simulink library "outp"  (R2021b)
(part 6 of 8)

      link override Signal_Limit/_maxval: Value=KOUTP_CCUAutoLampSts_flg_maxval
      link override Signal_Limit/_minval: Value=KOUTP_CCUAutoLampSts_flg_minval
      link override Signal_Override/_ovrdflg: Value=KOUTP_CCUAutoLampSts_flg_ovrdflg
      link override Signal_Override/_ovrdval: Value=KOUTP_CCUAutoLampSts_flg_ovrdval
  VTHC_CCUSyncLampSts_flg_Inproc : FVT_lib/outp/OverrideAndLimit  SystemSampleTime=-1  VariantActivationTime=update diagram  Latency=0  AutoFrameSizeCalculation=off
      link override Signal_Limit/_maxval: Value=KOUTP_CCUSyncLampSts_flg_maxval
      link override Signal_Limit/_minval: Value=KOUTP_CCUSyncLampSts_flg_minval
      link override Signal_Override/_ovrdflg: Value=KOUTP_CCUSyncLampSts_flg_ovrdflg
      link override Signal_Override/_ovrdval: Value=KOUTP_CCUSyncLampSts_flg_ovrdval
  VTHC_CCUSyncSts_flg_Inproc : FVT_lib/outp/OverrideAndLimit  SystemSampleTime=-1  VariantActivationTime=update diagram  Latency=0  AutoFrameSizeCalculation=off
      link override Signal_Limit/_maxval: Value=KOUTP_CCUSyncSts_flg_maxval
      link override Signal_Limit/_minval: Value=KOUTP_CCUSyncSts_flg_minval
      link override Signal_Override/_ovrdflg: Value=KOUTP_CCUSyncSts_flg_ovrdflg
      link override Signal_Override/_ovrdval: Value=KOUTP_CCUSyncSts_flg_ovrdval
  VTHC_CLVentEN_flg_Inproc : FVT_lib/outp/OverrideAndLimit  SystemSampleTime=-1  VariantActivationTime=update diagram  Latency=0  AutoFrameSizeCalculation=off
      link override Signal_Limit/_maxval: Value=KOUTP_CLVentEN_flg_maxval
      link override Signal_Limit/_minval: Value=KOUTP_CLVentEN_flg_minval
      link override Signal_Override/_ovrdflg: Value=KOUTP_CLVentEN_flg_ovrdflg
      link override Signal_Override/_ovrdval: Value=KOUTP_CLVentEN_flg_ovrdval
  VTHC_CRVentEN_flg_Inproc : FVT_lib/outp/OverrideAndLimit  SystemSampleTime=-1  VariantActivationTime=update diagram  Latency=0  AutoFrameSizeCalculation=off
      link override Signal_Limit/_maxval: Value=KOUTP_CRVentEN_flg_maxval
      link override Signal_Limit/_minval: Value=KOUTP_CRVentEN_flg_minval
      link override Signal_Override/_ovrdflg: Value=KOUTP_CRVentEN_flg_ovrdflg
      link override Signal_Override/_ovrdval: Value=KOUTP_CRVentEN_flg_ovrdval
  VTHC_CabinMode_enum_Inproc : FVT_lib/outp/OverrideAndLimit  SystemSampleTime=-1  VariantActivationTime=update diagram  Latency=0  AutoFrameSizeCalculation=off
      link override Signal_Limit/_maxval: Value=KOUTP_CabinMode_enum_maxval
      link override Signal_Limit/_minval: Value=KOUTP_CabinMode_enum_minval
      link override Signal_Override/_ovrdflg: Value=KOUTP_CabinMode_enum_ovrdflg
      link override Signal_Override/_ovrdval: Value=KOUTP_CabinMode_enum_ovrdval
  VTHC_CoolgFanActDuty_pct_Inproc : FVT_lib/outp/OverrideAndLimit  SystemSampleTime=-1  VariantActivationTime=update diagram  Latency=0  AutoFrameSizeCalculation=off
      link override Signal_Limit/_maxval: Value=KOUTP_CoolgFanActDuty_pct_maxval
      link override Signal_Limit/_minval: Value=KOUTP_CoolgFanActDuty_pct_minval
      link override Signal_Override/_ovrdflg: Value=KOUTP_CoolgFanActDuty_pct_ovrdflg
      link override Signal_Override/_ovrdval: Value=KOUTP_CoolgFanActDuty_pct_ovrdval
  VTHC_DrVentEN_flg_Inproc : FVT_lib/outp/OverrideAndLimit  SystemSampleTime=-1  VariantActivationTime=update diagram  Latency=0  AutoFrameSizeCalculation=off
      link override Signal_Limit/_maxval: Value=KOUTP_DrVentEN_flg_maxval
      link override Signal_Limit/_minval: Value=KOUTP_DrVentEN_flg_minval
      link override Signal_Override/_ovrdflg: Value=KOUTP_DrVentEN_flg_ovrdflg
      link override Signal_Override/_ovrdval: Value=KOUTP_DrVentEN_flg_ovrdval
  VTHC_EDriveMode_enum_Inproc : FVT_lib/outp/OverrideAndLimit  SystemSampleTime=-1  VariantActivationTime=update diagram  Latency=0  AutoFrameSizeCalculation=off
      link override Signal_Limit/_maxval: Value=KOUTP_EDriveMode_enum_maxval
      link override Signal_Limit/_minval: Value=KOUTP_EDriveMode_enum_minval
      link override Signal_Override/_ovrdflg: Value=KOUTP_EDriveMode_enum_ovrdflg
      link override Signal_Override/_ovrdval: Value=KOUTP_EDriveMode_enum_ovrdval
  VTHC_FDAGSCmd_enum_Inproc : FVT_lib/outp/OverrideAndLimit  SystemSampleTime=-1  VariantActivationTime=update diagram  Latency=0  AutoFrameSizeCalculation=off
      link override Signal_Limit/_maxval: Value=KOUTP_FDAGSCmd_enum_maxval
      link override Signal_Limit/_minval: Value=KOUTP_FDAGSCmd_enum_minval
      link override Signal_Override/_ovrdflg: Value=KOUTP_FDAGSCmd_enum_ovrdflg
      link override Signal_Override/_ovrdval: Value=KOUTP_FDAGSCmd_enum_ovrdval
  VTHC_FDBlowerCmd_pct_Inproc : FVT_lib/outp/OverrideAndLimit  SystemSampleTime=-1  VariantActivationTime=update diagram  Latency=0  AutoFrameSizeCalculation=off
      link override Signal_Limit/_maxval: Value=KOUTP_FDBlowerCmd_pct_maxval
      link override Signal_Limit/_minval: Value=KOUTP_FDBlowerCmd_pct_minval
      link override Signal_Override/_ovrdflg: Value=KOUTP_FDBlowerCmd_pct_ovrdflg
      link override Signal_Override/_ovrdval: Value=KOUTP_FDBlowerCmd_pct_ovrdval
  VTHC_FDCFGSAirIntCmd_enum_Inproc : FVT_lib/outp/OverrideAndLimit  SystemSampleTime=-1  VariantActivationTime=update diagram  Latency=0  AutoFrameSizeCalculation=off
      link override Signal_Limit/_maxval: Value=KOUTP_FDCFGSAirIntCmd_enum_maxval
      link override Signal_Limit/_minval: Value=KOUTP_FDCFGSAirIntCmd_enum_minval
      link override Signal_Override/_ovrdflg: Value=KOUTP_FDCFGSAirIntCmd_enum_ovrdflg
      link override Signal_Override/_ovrdval: Value=KOUTP_FDCFGSAirIntCmd_enum_ovrdval
  VTHC_FDCFGSAirIntSta_enum_Inproc : FVT_lib/outp/OverrideAndLimit  SystemSampleTime=-1  VariantActivationTime=update diagram  Latency=0  AutoFrameSizeCalculation=off
      link override Signal_Limit/_maxval: Value=KOUTP_FDCFGSAirIntSta_enum_maxval
      link override Signal_Limit/_minval: Value=KOUTP_FDCFGSAirIntSta_enum_minval
      link override Signal_Override/_ovrdflg: Value=KOUTP_FDCFGSAirIntSta_enum_ovrdflg
      link override Signal_Override/_ovrdval: Value=KOUTP_FDCFGSAirIntSta_enum_ovrdval
  VTHC_FDCFGSChCmd_enum_Inproc : FVT_lib/outp/OverrideAndLimit  SystemSampleTime=-1  VariantActivationTime=update diagram  Latency=0  AutoFrameSizeCalculation=off
      link override Signal_Limit/_maxval: Value=KOUTP_FDCFGSChCmd_enum_maxval
      link override Signal_Limit/_minval: Value=KOUTP_FDCFGSChCmd_enum_minval
      link override Signal_Override/_ovrdflg: Value=KOUTP_FDCFGSChCmd_enum_ovrdflg
      link override Signal_Override/_ovrdval: Value=KOUTP_FDCFGSChCmd_enum_ovrdval
  VTHC_FDCFGSChSta_enum_Inproc : FVT_lib/outp/OverrideAndLimit  SystemSampleTime=-1  VariantActivationTime=update diagram  Latency=0  AutoFrameSizeCalculation=off
      link override Signal_Limit/_maxval: Value=KOUTP_FDCFGSChSta_enum_maxval
      link override Signal_Limit/_minval: Value=KOUTP_FDCFGSChSta_enum_minval
      link override Signal_Override/_ovrdflg: Value=KOUTP_FDCFGSChSta_enum_ovrdflg
      link override Signal_Override/_ovrdval: Value=KOUTP_FDCFGSChSta_enum_ovrdval
  VTHC_FDCFGSFuncSta_flg_Inproc : FVT_lib/outp/OverrideAndLimit  SystemSampleTime=-1  VariantActivationTime=update diagram  Latency=0  AutoFrameSizeCalculation=off
      link override Signal_Limit/_maxval: Value=KOUTP_FDCFGSFuncSta_flg_maxval
      link override Signal_Limit/_minval: Value=KOUTP_FDCFGSFuncSta_flg_minval
      link override Signal_Override/_ovrdflg: Value=KOUTP_FDCFGSFuncSta_flg_ovrdflg
      link override Signal_Override/_ovrdval: Value=KOUTP_FDCFGSFuncSta_flg_ovrdval
  VTHC_FDCFGSIONCmd_flg_Inproc : FVT_lib/outp/OverrideAndLimit  SystemSampleTime=-1  VariantActivationTime=update diagram  Latency=0  AutoFrameSizeCalculation=off
      link override Signal_Limit/_maxval: Value=KOUTP_FDCFGSIONCmd_flg_maxval
      link override Signal_Limit/_minval: Value=KOUTP_FDCFGSIONCmd_flg_minval
      link override Signal_Override/_ovrdflg: Value=KOUTP_FDCFGSIONCmd_flg_ovrdflg
      link override Signal_Override/_ovrdval: Value=KOUTP_FDCFGSIONCmd_flg_ovrdval
  VTHC_FDCFGSIONSWSta_flg_Inproc : FVT_lib/outp/OverrideAndLimit  SystemSampleTime=-1  VariantActivationTime=update diagram  Latency=0  AutoFrameSizeCalculation=off
      link override Signal_Limit/_maxval: Value=KOUTP_FDCFGSIONSWSta_flg_maxval
      link override Signal_Limit/_minval: Value=KOUTP_FDCFGSIONSWSta_flg_minval
      link override Signal_Override/_ovrdflg: Value=KOUTP_FDCFGSIONSWSta_flg_ovrdflg
      link override Signal_Override/_ovrdval: Value=KOUTP_FDCFGSIONSWSta_flg_ovrdval
  VTHC_FDCFGSLearnCmd_enum_Inproc : FVT_lib/outp/OverrideAndLimit  SystemSampleTime=-1  VariantActivationTime=update diagram  Latency=0  AutoFrameSizeCalculation=off
      link override Signal_Limit/_maxval: Value=KOUTP_FDCFGSLearnCmd_enum_maxval
      link override Signal_Limit/_minval: Value=KOUTP_FDCFGSLearnCmd_enum_minval
      link override Signal_Override/_ovrdflg: Value=KOUTP_FDCFGSLearnCmd_enum_ovrdflg
      link override Signal_Override/_ovrdval: Value=KOUTP_FDCFGSLearnCmd_enum_ovrdval
  VTHC_FDCTHCAirIntZ3Sta_enum_Inproc : FVT_lib/outp/OverrideAndLimit  SystemSampleTime=-1  VariantActivationTime=update diagram  Latency=0  AutoFrameSizeCalculation=off
      link override Signal_Limit/_maxval: Value=KOUTP_FDCTHCAirIntZ3Sta_enum_maxval
      link override Signal_Limit/_minval: Value=KOUTP_FDCTHCAirIntZ3Sta_enum_minval
      link override Signal_Override/_ovrdflg: Value=KOUTP_FDCTHCAirIntZ3Sta_enum_ovrdflg
      link override Signal_Override/_ovrdval: Value=KOUTP_FDCTHCAirIntZ3Sta_enum_ovrdval
  VTHC_FDCTHCCLEVentYSta_enum_Inproc : FVT_lib/outp/OverrideAndLimit  SystemSampleTime=-1  VariantActivationTime=update diagram  Latency=0  AutoFrameSizeCalculation=off
      link override Signal_Limit/_maxval: Value=KOUTP_FDCTHCCLEVentYSta_enum_maxval
      link override Signal_Limit/_minval: Value=KOUTP_FDCTHCCLEVentYSta_enum_minval
      link override Signal_Override/_ovrdflg: Value=KOUTP_FDCTHCCLEVentYSta_enum_ovrdflg
      link override Signal_Override/_ovrdval: Value=KOUTP_FDCTHCCLEVentYSta_enum_ovrdval
  VTHC_FDCTHCCLEVentZSta_enum_Inproc : FVT_lib/outp/OverrideAndLimit  SystemSampleTime=-1  VariantActivationTime=update diagram  Latency=0  AutoFrameSizeCalculation=off
      link override Signal_Limit/_maxval: Value=KOUTP_FDCTHCCLEVentZSta_enum_maxval
      link override Signal_Limit/_minval: Value=KOUTP_FDCTHCCLEVentZSta_enum_minval
      link override Signal_Override/_ovrdflg: Value=KOUTP_FDCTHCCLEVentZSta_enum_ovrdflg
      link override Signal_Override/_ovrdval: Value=KOUTP_FDCTHCCLEVentZSta_enum_ovrdval
  VTHC_FDCTHCCLVentENSta_flg_Inproc : FVT_lib/outp/OverrideAndLimit  SystemSampleTime=-1  VariantActivationTime=update diagram  Latency=0  AutoFrameSizeCalculation=off
      link override Signal_Limit/_maxval: Value=KOUTP_FDCTHCCLVentENSta_flg_maxval
      link override Signal_Limit/_minval: Value=KOUTP_FDCTHCCLVentENSta_flg_minval
      link override Signal_Override/_ovrdflg: Value=KOUTP_FDCTHCCLVentENSta_flg_ovrdflg
      link override Signal_Override/_ovrdval: Value=KOUTP_FDCTHCCLVentENSta_flg_ovrdval
  VTHC_FDCTHCCREVentYSta_enum_Inproc : FVT_lib/outp/OverrideAndLimit  SystemSampleTime=-1  VariantActivationTime=update diagram  Latency=0  AutoFrameSizeCalculation=off
      link override Signal_Limit/_maxval: Value=KOUTP_FDCTHCCREVentYSta_enum_maxval
      link override Signal_Limit/_minval: Value=KOUTP_FDCTHCCREVentYSta_enum_minval
      link override Signal_Override/_ovrdflg: Value=KOUTP_FDCTHCCREVentYSta_enum_ovrdflg
      link override Signal_Override/_ovrdval: Value=KOUTP_FDCTHCCREVentYSta_enum_ovrdval
  VTHC_FDCTHCCREVentZSta_enum_Inproc : FVT_lib/outp/OverrideAndLimit  SystemSampleTime=-1  VariantActivationTime=update diagram  Latency=0  AutoFrameSizeCalculation=off
      link override Signal_Limit/_maxval: Value=KOUTP_FDCTHCCREVentZSta_enum_maxval
      link override Signal_Limit/_minval: Value=KOUTP_FDCTHCCREVentZSta_enum_minval
      link override Signal_Override/_ovrdflg: Value=KOUTP_FDCTHCCREVentZSta_enum_ovrdflg
      link override Signal_Override/_ovrdval: Value=KOUTP_FDCTHCCREVentZSta_enum_ovrdval
  VTHC_FDCTHCCRVentENSta_flg_Inproc : FVT_lib/outp/OverrideAndLimit  SystemSampleTime=-1  VariantActivationTime=update diagram  Latency=0  AutoFrameSizeCalculation=off
      link override Signal_Limit/_maxval: Value=KOUTP_FDCTHCCRVentENSta_flg_maxval
      link override Signal_Limit/_minval: Value=KOUTP_FDCTHCCRVentENSta_flg_minval
      link override Signal_Override/_ovrdflg: Value=KOUTP_FDCTHCCRVentENSta_flg_ovrdflg
      link override Signal_Override/_ovrdval: Value=KOUTP_FDCTHCCRVentENSta_flg_ovrdval
  VTHC_FDCTHCDrEVentModeSta_enum_Inproc : FVT_lib/outp/OverrideAndLimit  SystemSampleTime=-1  VariantActivationTime=update diagram  Latency=0  AutoFrameSizeCalculation=off
      link override Signal_Limit/_maxval: Value=KOUTP_FDCTHCDrEVentModeSta_enum_maxval
      link override Signal_Limit/_minval: Value=KOUTP_FDCTHCDrEVentModeSta_enum_minval
      link override Signal_Override/_ovrdflg: Value=KOUTP_FDCTHCDrEVentModeSta_enum_ovrdflg
      link override Signal_Override/_ovrdval: Value=KOUTP_FDCTHCDrEVentModeSta_enum_ovrdval
  VTHC_FDCTHCDrEVentYSta_enum_Inproc : FVT_lib/outp/OverrideAndLimit  SystemSampleTime=-1  VariantActivationTime=update diagram  Latency=0  AutoFrameSizeCalculation=off
      link override Signal_Limit/_maxval: Value=KOUTP_FDCTHCDrEVentYSta_enum_maxval
      link override Signal_Limit/_minval: Value=KOUTP_FDCTHCDrEVentYSta_enum_minval
      link override Signal_Override/_ovrdflg: Value=KOUTP_FDCTHCDrEVentYSta_enum_ovrdflg
      link override Signal_Override/_ovrdval: Value=KOUTP_FDCTHCDrEVentYSta_enum_ovrdval
  VTHC_FDCTHCDrEVentZSta_enum_Inproc : FVT_lib/outp/OverrideAndLimit  SystemSampleTime=-1  VariantActivationTime=update diagram  Latency=0  AutoFrameSizeCalculation=off
      link override Signal_Limit/_maxval: Value=KOUTP_FDCTHCDrEVentZSta_enum_maxval
      link override Signal_Limit/_minval: Value=KOUTP_FDCTHCDrEVentZSta_enum_minval
      link override Signal_Override/_ovrdflg: Value=KOUTP_FDCTHCDrEVentZSta_enum_ovrdflg
      link override Signal_Override/_ovrdval: Value=KOUTP_FDCTHCDrEVentZSta_enum_ovrdval
  VTHC_FDCTHCDrVentENSta_flg_Inproc : FVT_lib/outp/OverrideAndLimit  SystemSampleTime=-1  VariantActivationTime=update diagram  Latency=0  AutoFrameSizeCalculation=off
      link override Signal_Limit/_maxval: Value=KOUTP_FDCTHCDrVentENSta_flg_maxval
      link override Signal_Limit/_minval: Value=KOUTP_FDCTHCDrVentENSta_flg_minval
      link override Signal_Override/_ovrdflg: Value=KOUTP_FDCTHCDrVentENSta_flg_ovrdflg
      link override Signal_Override/_ovrdval: Value=KOUTP_FDCTHCDrVentENSta_flg_ovrdval
  VTHC_FDCTHCMAPTCForceOFFSta_flg_Inproc : FVT_lib/outp/OverrideAndLimit  SystemSampleTime=-1  VariantActivationTime=update diagram  Latency=0  AutoFrameSizeCalculation=off
      link override Signal_Limit/_maxval: Value=KOUTP_FDCTHCMAPTCForceOFFSta_flg_maxval
      link override Signal_Limit/_minval: Value=KOUTP_FDCTHCMAPTCForceOFFSta_flg_minval
      link override Signal_Override/_ovrdflg: Value=KOUTP_FDCTHCMAPTCForceOFFSta_flg_ovrdflg
      link override Signal_Override/_ovrdval: Value=KOUTP_FDCTHCMAPTCForceOFFSta_flg_ovrdval
  VTHC_FDCTHCMPreWPTCHeatSta_enum_Inproc : FVT_lib/outp/OverrideAndLimit  SystemSampleTime=-1  VariantActivationTime=update diagram  Latency=0  AutoFrameSizeCalculation=off
      link override Signal_Limit/_maxval: Value=KOUTP_FDCTHCMPreWPTCHeatSta_enum_maxval
      link override Signal_Limit/_minval: Value=KOUTP_FDCTHCMPreWPTCHeatSta_enum_minval
      link override Signal_Override/_ovrdflg: Value=KOUTP_FDCTHCMPreWPTCHeatSta_enum_ovrdflg
      link override Signal_Override/_ovrdval: Value=KOUTP_FDCTHCMPreWPTCHeatSta_enum_ovrdval
  VTHC_FDCTHCPsEVentModeSta_enum_Inproc : FVT_lib/outp/OverrideAndLimit  SystemSampleTime=-1  VariantActivationTime=update diagram  Latency=0  AutoFrameSizeCalculation=off
      link override Signal_Limit/_maxval: Value=KOUTP_FDCTHCPsEVentModeSta_enum_maxval
      link override Signal_Limit/_minval: Value=KOUTP_FDCTHCPsEVentModeSta_enum_minval
      link override Signal_Override/_ovrdflg: Value=KOUTP_FDCTHCPsEVentModeSta_enum_ovrdflg
      link override Signal_Override/_ovrdval: Value=KOUTP_FDCTHCPsEVentModeSta_enum_ovrdval
  VTHC_FDCTHCPsEVentYSta_enum_Inproc : FVT_lib/outp/OverrideAndLimit  SystemSampleTime=-1  VariantActivationTime=update diagram  Latency=0  AutoFrameSizeCalculation=off
      link override Signal_Limit/_maxval: Value=KOUTP_FDCTHCPsEVentYSta_enum_maxval
      link override Signal_Limit/_minval: Value=KOUTP_FDCTHCPsEVentYSta_enum_minval
      link override Signal_Override/_ovrdflg: Value=KOUTP_FDCTHCPsEVentYSta_enum_ovrdflg
      link override Signal_Override/_ovrdval: Value=KOUTP_FDCTHCPsEVentYSta_enum_ovrdval
  VTHC_FDCTHCPsEVentZSta_enum_Inproc : FVT_lib/outp/OverrideAndLimit  SystemSampleTime=-1  VariantActivationTime=update diagram  Latency=0  AutoFrameSizeCalculation=off
      link override Signal_Limit/_maxval: Value=KOUTP_FDCTHCPsEVentZSta_enum_maxval
      link override Signal_Limit/_minval: Value=KOUTP_FDCTHCPsEVentZSta_enum_minval
      link override Signal_Override/_ovrdflg: Value=KOUTP_FDCTHCPsEVentZSta_enum_ovrdflg
      link override Signal_Override/_ovrdval: Value=KOUTP_FDCTHCPsEVentZSta_enum_ovrdval
  VTHC_FDCTHCPsVentENSta_flg_Inproc : FVT_lib/outp/OverrideAndLimit  SystemSampleTime=-1  VariantActivationTime=update diagram  Latency=0  AutoFrameSizeCalculation=off
      link override Signal_Limit/_maxval: Value=KOUTP_FDCTHCPsVentENSta_flg_maxval
      link override Signal_Limit/_minval: Value=KOUTP_FDCTHCPsVentENSta_flg_minval
      link override Signal_Override/_ovrdflg: Value=KOUTP_FDCTHCPsVentENSta_flg_ovrdflg
      link override Signal_Override/_ovrdval: Value=KOUTP_FDCTHCPsVentENSta_flg_ovrdval
  VTHC_FDCompCmd_rpm_Inproc : FVT_lib/outp/OverrideAndLimit  SystemSampleTime=-1  VariantActivationTime=update diagram  Latency=0  AutoFrameSizeCalculation=off
      link override Signal_Limit/_maxval: Value=KOUTP_FDCompCmd_rpm_maxval
      link override Signal_Limit/_minval: Value=KOUTP_FDCompCmd_rpm_minval
      link override Signal_Override/_ovrdflg: Value=KOUTP_FDCompCmd_rpm_ovrdflg
      link override Signal_Override/_ovrdval: Value=KOUTP_FDCompCmd_rpm_ovrdval
  VTHC_FDEWP1Cmd_enum_Inproc : FVT_lib/outp/OverrideAndLimit  SystemSampleTime=-1  VariantActivationTime=update diagram  Latency=0  AutoFrameSizeCalculation=off
      link override Signal_Limit/_maxval: Value=KOUTP_FDEWP1Cmd_enum_maxval
      link override Signal_Limit/_minval: Value=KOUTP_FDEWP1Cmd_enum_minval
      link override Signal_Override/_ovrdflg: Value=KOUTP_FDEWP1Cmd_enum_ovrdflg
      link override Signal_Override/_ovrdval: Value=KOUTP_FDEWP1Cmd_enum_ovrdval
  VTHC_FDEWP2Cmd_enum_Inproc : FVT_lib/outp/OverrideAndLimit  SystemSampleTime=-1  VariantActivationTime=update diagram  Latency=0  AutoFrameSizeCalculation=off
      link override Signal_Limit/_maxval: Value=KOUTP_FDEWP2Cmd_enum_maxval
      link override Signal_Limit/_minval: Value=KOUTP_FDEWP2Cmd_enum_minval
      link override Signal_Override/_ovrdflg: Value=KOUTP_FDEWP2Cmd_enum_ovrdflg
      link override Signal_Override/_ovrdval: Value=KOUTP_FDEWP2Cmd_enum_ovrdval
  VTHC_FDEWP3Cmd_enum_Inproc : FVT_lib/outp/OverrideAndLimit  SystemSampleTime=-1  VariantActivationTime=update diagram  Latency=0  AutoFrameSizeCalculation=off
      link override Signal_Limit/_maxval: Value=KOUTP_FDEWP3Cmd_enum_maxval
      link override Signal_Limit/_minval: Value=KOUTP_FDEWP3Cmd_enum_minval
      link override Signal_Override/_ovrdflg: Value=KOUTP_FDEWP3Cmd_enum_ovrdflg
      link override Signal_Override/_ovrdval: Value=KOUTP_FDEWP3Cmd_enum_ovrdval
  VTHC_FDEXV1Cmd_step_Inproc : FVT_lib/outp/OverrideAndLimit  SystemSampleTime=-1  VariantActivationTime=update diagram  Latency=0  AutoFrameSizeCalculation=off
      link override Signal_Limit/_maxval: Value=KOUTP_FDEXV1Cmd_step_maxval
      link override Signal_Limit/_minval: Value=KOUTP_FDEXV1Cmd_step_minval
      link override Signal_Override/_ovrdflg: Value=KOUTP_FDEXV1Cmd_step_ovrdflg
      link override Signal_Override/_ovrdval: Value=KOUTP_FDEXV1Cmd_step_ovrdval
  VTHC_FDEXV2Cmd_step_Inproc : FVT_lib/outp/OverrideAndLimit  SystemSampleTime=-1  VariantActivationTime=update diagram  Latency=0  AutoFrameSizeCalculation=off
      link override Signal_Limit/_maxval: Value=KOUTP_FDEXV2Cmd_step_maxval
      link override Signal_Limit/_minval: Value=KOUTP_FDEXV2Cmd_step_minval
      link override Signal_Override/_ovrdflg: Value=KOUTP_FDEXV2Cmd_step_ovrdflg
      link override Signal_Override/_ovrdval: Value=KOUTP_FDEXV2Cmd_step_ovrdval
  VTHC_FDFWVCmd_flg_Inproc : FVT_lib/outp/OverrideAndLimit  SystemSampleTime=-1  VariantActivationTime=update diagram  Latency=0  AutoFrameSizeCalculation=off
      link override Signal_Limit/_maxval: Value=KOUTP_FDFWVCmd_flg_maxval
      link override Signal_Limit/_minval: Value=KOUTP_FDFWVCmd_flg_minval
      link override Signal_Override/_ovrdflg: Value=KOUTP_FDFWVCmd_flg_ovrdflg
      link override Signal_Override/_ovrdval: Value=KOUTP_FDFWVCmd_flg_ovrdval
  VTHC_FDFrLeAPTCHeatPwrCmd_W_Inproc : FVT_lib/outp/OverrideAndLimit  SystemSampleTime=-1  VariantActivationTime=update diagram  Latency=0  AutoFrameSizeCalculation=off
      link override Signal_Limit/_maxval: Value=KOUTP_FDFrLeAPTCHeatPwrCmd_W_maxval
      link override Signal_Limit/_minval: Value=KOUTP_FDFrLeAPTCHeatPwrCmd_W_minval
      link override Signal_Override/_ovrdflg: Value=KOUTP_FDFrLeAPTCHeatPwrCmd_W_ovrdflg
      link override Signal_Override/_ovrdval: Value=KOUTP_FDFrLeAPTCHeatPwrCmd_W_ovrdval
  VTHC_FDFrRiAPTCHeatPwrCmd_W_Inproc : FVT_lib/outp/OverrideAndLimit  SystemSampleTime=-1  VariantActivationTime=update diagram  Latency=0  AutoFrameSizeCalculation=off
      link override Signal_Limit/_maxval: Value=KOUTP_FDFrRiAPTCHeatPwrCmd_W_maxval
      link override Signal_Limit/_minval: Value=KOUTP_FDFrRiAPTCHeatPwrCmd_W_minval
      link override Signal_Override/_ovrdflg: Value=KOUTP_FDFrRiAPTCHeatPwrCmd_W_ovrdflg
      link override Signal_Override/_ovrdval: Value=KOUTP_FDFrRiAPTCHeatPwrCmd_W_ovrdval
  VTHC_FDFrWPTCHeatPwrCmd_W_Inproc : FVT_lib/outp/OverrideAndLimit  SystemSampleTime=-1  VariantActivationTime=update diagram  Latency=0  AutoFrameSizeCalculation=off
      link override Signal_Limit/_maxval: Value=KOUTP_FDFrWPTCHeatPwrCmd_W_maxval
      link override Signal_Limit/_minval: Value=KOUTP_FDFrWPTCHeatPwrCmd_W_minval
      link override Signal_Override/_ovrdflg: Value=KOUTP_FDFrWPTCHeatPwrCmd_W_ovrdflg
      link override Signal_Override/_ovrdval: Value=KOUTP_FDFrWPTCHeatPwrCmd_W_ovrdval
  VTHC_FDRecyAutoCmd_enum_Inproc : FVT_lib/outp/OverrideAndLimit  SystemSampleTime=-1  VariantActivationTime=update diagram  Latency=0  AutoFrameSizeCalculation=off
      link override Signal_Limit/_maxval: Value=KOUTP_FDRecyAutoCmd_enum_maxval
      link override Signal_Limit/_minval: Value=KOUTP_FDRecyAutoCmd_enum_minval
      link override Signal_Override/_ovrdflg: Value=KOUTP_FDRecyAutoCmd_enum_ovrdflg
      link override Signal_Override/_ovrdval: Value=KOUTP_FDRecyAutoCmd_enum_ovrdval
  VTHC_FDRrAPTCHeatPwrCmd_W_Inproc : FVT_lib/outp/OverrideAndLimit  SystemSampleTime=-1  VariantActivationTime=update diagram  Latency=0  AutoFrameSizeCalculation=off
      link override Signal_Limit/_maxval: Value=KOUTP_FDRrAPTCHeatPwrCmd_W_maxval
      link override Signal_Limit/_minval: Value=KOUTP_FDRrAPTCHeatPwrCmd_W_minval
      link override Signal_Override/_ovrdflg: Value=KOUTP_FDRrAPTCHeatPwrCmd_W_ovrdflg
      link override Signal_Override/_ovrdval: Value=KOUTP_FDRrAPTCHeatPwrCmd_W_ovrdval
  VTHC_FDSOTXVCmd_flg_Inproc : FVT_lib/outp/OverrideAndLimit  SystemSampleTime=-1  VariantActivationTime=update diagram  Latency=0  AutoFrameSizeCalculation=off
      link override Signal_Limit/_maxval: Value=KOUTP_FDSOTXVCmd_flg_maxval
      link override Signal_Limit/_minval: Value=KOUTP_FDSOTXVCmd_flg_minval
      link override Signal_Override/_ovrdflg: Value=KOUTP_FDSOTXVCmd_flg_ovrdflg
      link override Signal_Override/_ovrdval: Value=KOUTP_FDSOTXVCmd_flg_ovrdval
  VTHC_FDSOV1Cmd_flg_Inproc : FVT_lib/outp/OverrideAndLimit  SystemSampleTime=-1  VariantActivationTime=update diagram  Latency=0  AutoFrameSizeCalculation=off
      link override Signal_Limit/_maxval: Value=KOUTP_FDSOV1Cmd_flg_maxval
      link override Signal_Limit/_minval: Value=KOUTP_FDSOV1Cmd_flg_minval
      link override Signal_Override/_ovrdflg: Value=KOUTP_FDSOV1Cmd_flg_ovrdflg
      link override Signal_Override/_ovrdval: Value=KOUTP_FDSOV1Cmd_flg_ovrdval
  VTHC_FDSOV2Cmd_flg_Inproc : FVT_lib/outp/OverrideAndLimit  SystemSampleTime=-1  VariantActivationTime=update diagram  Latency=0  AutoFrameSizeCalculation=off
      link override Signal_Limit/_maxval: Value=KOUTP_FDSOV2Cmd_flg_maxval
      link override Signal_Limit/_minval: Value=KOUTP_FDSOV2Cmd_flg_minval
      link override Signal_Override/_ovrdflg: Value=KOUTP_FDSOV2Cmd_flg_ovrdflg
      link override Signal_Override/_ovrdval: Value=KOUTP_FDSOV2Cmd_flg_ovrdval
  VTHC_FDSOV3Cmd_flg_Inproc : FVT_lib/outp/OverrideAndLimit  SystemSampleTime=-1  VariantActivationTime=update diagram  Latency=0  AutoFrameSizeCalculation=off
      link override Signal_Limit/_maxval: Value=KOUTP_FDSOV3Cmd_flg_maxval
      link override Signal_Limit/_minval: Value=KOUTP_FDSOV3Cmd_flg_minval
      link override Signal_Override/_ovrdflg: Value=KOUTP_FDSOV3Cmd_flg_ovrdflg
      link override Signal_Override/_ovrdval: Value=KOUTP_FDSOV3Cmd_flg_ovrdval
  VTHC_FDTWVCmd_pct_Inproc : FVT_lib/outp/OverrideAndLimit  SystemSampleTime=-1  VariantActivationTime=update diagram  Latency=0  AutoFrameSizeCalculation=off
      link override Signal_Limit/_maxval: Value=KOUTP_FDTWVCmd_pct_maxval
      link override Signal_Limit/_minval: Value=KOUTP_FDTWVCmd_pct_minval
      link override Signal_Override/_ovrdflg: Value=KOUTP_FDTWVCmd_pct_ovrdflg
      link override Signal_Override/_ovrdval: Value=KOUTP_FDTWVCmd_pct_ovrdval
  VTHC_FaceM_flg_Inproc : FVT_lib/outp/OverrideAndLimit  SystemSampleTime=-1  VariantActivationTime=update diagram  Latency=0  AutoFrameSizeCalculation=off
      link override Signal_Limit/_maxval: Value=KOUTP_FaceM_flg_maxval
      link override Signal_Limit/_minval: Value=KOUTP_FaceM_flg_minval
      link override Signal_Override/_ovrdflg: Value=KOUTP_FaceM_flg_ovrdflg
      link override Signal_Override/_ovrdval: Value=KOUTP_FaceM_flg_ovrdval
  VTHC_Face_flg_Inproc : FVT_lib/outp/OverrideAndLimit  SystemSampleTime=-1  VariantActivationTime=update diagram  Latency=0  AutoFrameSizeCalculation=off
      link override Signal_Limit/_maxval: Value=KOUTP_Face_flg_maxval
      link override Signal_Limit/_minval: Value=KOUTP_Face_flg_minval
      link override Signal_Override/_ovrdflg: Value=KOUTP_Face_flg_ovrdflg
      link override Signal_Override/_ovrdval: Value=KOUTP_Face_flg_ovrdval
  VTHC_FootM_flg_Inproc : FVT_lib/outp/OverrideAndLimit  SystemSampleTime=-1  VariantActivationTime=update diagram  Latency=0  AutoFrameSizeCalculation=off
      link override Signal_Limit/_maxval: Value=KOUTP_FootM_flg_maxval
      link override Signal_Limit/_minval: Value=KOUTP_FootM_flg_minval
      link override Signal_Override/_ovrdflg: Value=KOUTP_FootM_flg_ovrdflg
      link override Signal_Override/_ovrdval: Value=KOUTP_FootM_flg_ovrdval
  VTHC_Foot_flg_Inproc : FVT_lib/outp/OverrideAndLimit  SystemSampleTime=-1  VariantActivationTime=update diagram  Latency=0  AutoFrameSizeCalculation=off
      link override Signal_Limit/_maxval: Value=KOUTP_Foot_flg_maxval
      link override Signal_Limit/_minval: Value=KOUTP_Foot_flg_minval
      link override Signal_Override/_ovrdflg: Value=KOUTP_Foot_flg_ovrdflg
      link override Signal_Override/_ovrdval: Value=KOUTP_Foot_flg_ovrdval
  VTHC_Frost_flg_Inproc : FVT_lib/outp/OverrideAndLimit  SystemSampleTime=-1  VariantActivationTime=update diagram  Latency=0  AutoFrameSizeCalculation=off
      link override Signal_Limit/_maxval: Value=KOUTP_Frost_flg_maxval
      link override Signal_Limit/_minval: Value=KOUTP_Frost_flg_minval
      link override Signal_Override/_ovrdflg: Value=KOUTP_Frost_flg_ovrdflg
      link override Signal_Override/_ovrdval: Value=KOUTP_Frost_flg_ovrdval
  VTHC_PsVentEN_flg_Inproc : FVT_lib/outp/OverrideAndLimit  SystemSampleTime=-1  VariantActivationTime=update diagram  Latency=0  AutoFrameSizeCalculation=off
      link override Signal_Limit/_maxval: Value=KOUTP_PsVentEN_flg_maxval
      link override Signal_Limit/_minval: Value=KOUTP_PsVentEN_flg_minval
      link override Signal_Override/_ovrdflg: Value=KOUTP_PsVentEN_flg_ovrdflg
      link override Signal_Override/_ovrdval: Value=KOUTP_PsVentEN_flg_ovrdval
  VTHC_RecAutoFlg_flg_Inproc : FVT_lib/outp/OverrideAndLimit  SystemSampleTime=-1  VariantActivationTime=update diagram  Latency=0  AutoFrameSizeCalculation=off
      link override Signal_Limit/_maxval: Value=KOUTP_RecAutoFlg_flg_maxval
      link override Signal_Limit/_minval: Value=KOUTP_RecAutoFlg_flg_minval
      link override Signal_Override/_ovrdflg: Value=KOUTP_RecAutoFlg_flg_ovrdflg
      link override Signal_Override/_ovrdval: Value=KOUTP_RecAutoFlg_flg_ovrdval
  VTHC_fdefog_flg_Inproc : FVT_lib/outp/OverrideAndLimit  SystemSampleTime=-1  VariantActivationTime=update diagram  Latency=0  AutoFrameSizeCalculation=off
      link override Signal_Limit/_maxval: Value=KOUTP_fdefog_flg_maxval
      link override Signal_Limit/_minval: Value=KOUTP_fdefog_flg_minval
      link override Signal_Override/_ovrdflg: Value=KOUTP_fdefog_flg_ovrdflg
      link override Signal_Override/_ovrdval: Value=KOUTP_fdefog_flg_ovrdval
  VTHC_sigAirIntenZon1St_enum_Inproc : FVT_lib/outp/OverrideAndLimit  SystemSampleTime=-1  VariantActivationTime=update diagram  Latency=0  AutoFrameSizeCalculation=off
      link override Signal_Limit/_maxval: Value=KOUTP_sigAirIntenZon1St_enum_maxval
      link override Signal_Limit/_minval: Value=KOUTP_sigAirIntenZon1St_enum_minval
      link override Signal_Override/_ovrdflg: Value=KOUTP_sigAirIntenZon1St_enum_ovrdflg
      link override Signal_Override/_ovrdval: Value=KOUTP_sigAirIntenZon1St_enum_ovrdval
  VTHC_sigAmbAirT_C_Inproc : FVT_lib/outp/OverrideAndLimit  SystemSampleTime=-1  VariantActivationTime=update diagram  Latency=0  AutoFrameSizeCalculation=off
      link override Signal_Limit/_maxval: Value=KOUTP_sigAmbAirT_C_maxval
      link override Signal_Limit/_minval: Value=KOUTP_sigAmbAirT_C_minval
      link override Signal_Override/_ovrdflg: Value=KOUTP_sigAmbAirT_C_ovrdflg
      link override Signal_Override/_ovrdval: Value=KOUTP_sigAmbAirT_C_ovrdval
  VTHC_sigCbnAirT_C_Inproc : FVT_lib/outp/OverrideAndLimit  SystemSampleTime=-1  VariantActivationTime=update diagram  Latency=0  AutoFrameSizeCalculation=off
      link override Signal_Limit/_maxval: Value=KOUTP_sigCbnAirT_C_maxval
      link override Signal_Limit/_minval: Value=KOUTP_sigCbnAirT_C_minval
      link override Signal_Override/_ovrdflg: Value=KOUTP_sigCbnAirT_C_ovrdflg
      link override Signal_Override/_ovrdval: Value=KOUTP_sigCbnAirT_C_ovrdval
  VTHC_sigCbnSolarLeft_W_Inproc : FVT_lib/outp/OverrideAndLimit  SystemSampleTime=-1  VariantActivationTime=update diagram  Latency=0  AutoFrameSizeCalculation=off
      link override Signal_Limit/_maxval: Value=KOUTP_sigCbnSolarLeft_W_maxval
      link override Signal_Limit/_minval: Value=KOUTP_sigCbnSolarLeft_W_minval
      link override Signal_Override/_ovrdflg: Value=KOUTP_sigCbnSolarLeft_W_ovrdflg
      link override Signal_Override/_ovrdval: Value=KOUTP_sigCbnSolarLeft_W_ovrdval
  VTHC_sigCbnSolarRight_W_Inproc : FVT_lib/outp/OverrideAndLimit  SystemSampleTime=-1  VariantActivationTime=update diagram  Latency=0  AutoFrameSizeCalculation=off
      link override Signal_Limit/_maxval: Value=KOUTP_sigCbnSolarRight_W_maxval
      link override Signal_Limit/_minval: Value=KOUTP_sigCbnSolarRight_W_minval
      link override Signal_Override/_ovrdflg: Value=KOUTP_sigCbnSolarRight_W_ovrdflg
      link override Signal_Override/_ovrdval: Value=KOUTP_sigCbnSolarRight_W_ovrdval
  VTHC_sigClntTHvBattIn_C_Inproc : FVT_lib/outp/OverrideAndLimit  SystemSampleTime=-1  VariantActivationTime=update diagram  Latency=0  AutoFrameSizeCalculation=off
      link override Signal_Limit/_maxval: Value=KOUTP_sigClntTHvBattIn_C_maxval
      link override Signal_Limit/_minval: Value=KOUTP_sigClntTHvBattIn_C_minval
      link override Signal_Override/_ovrdflg: Value=KOUTP_sigClntTHvBattIn_C_ovrdflg
      link override Signal_Override/_ovrdval: Value=KOUTP_sigClntTHvBattIn_C_ovrdval
  VTHC_sigClntTHvBattOut_C_Inproc : FVT_lib/outp/OverrideAndLimit  SystemSampleTime=-1  VariantActivationTime=update diagram  Latency=0  AutoFrameSizeCalculation=off
      link override Signal_Limit/_maxval: Value=KOUTP_sigClntTHvBattOut_C_maxval
      link override Signal_Limit/_minval: Value=KOUTP_sigClntTHvBattOut_C_minval
      link override Signal_Override/_ovrdflg: Value=KOUTP_sigClntTHvBattOut_C_ovrdflg
      link override Signal_Override/_ovrdval: Value=KOUTP_sigClntTHvBattOut_C_ovrdval
  VTHC_sigDfrstSt_flg_Inproc : FVT_lib/outp/OverrideAndLimit  SystemSampleTime=-1  VariantActivationTime=update diagram  Latency=0  AutoFrameSizeCalculation=off
      link override Signal_Limit/_maxval: Value=KOUTP_sigDfrstSt_flg_maxval
      link override Signal_Limit/_minval: Value=KOUTP_sigDfrstSt_flg_minval
      link override Signal_Override/_ovrdflg: Value=KOUTP_sigDfrstSt_flg_ovrdflg
      link override Signal_Override/_ovrdval: Value=KOUTP_sigDfrstSt_flg_ovrdval
  VTHC_sigRecircSt_flg_Inproc : FVT_lib/outp/OverrideAndLimit  SystemSampleTime=-1  VariantActivationTime=update diagram  Latency=0  AutoFrameSizeCalculation=off
      link override Signal_Limit/_maxval: Value=KOUTP_sigRecircSt_flg_maxval
      link override Signal_Limit/_minval: Value=KOUTP_sigRecircSt_flg_minval
      link override Signal_Override/_ovrdflg: Value=KOUTP_sigRecircSt_flg_ovrdflg
      link override Signal_Override/_ovrdval: Value=KOUTP_sigRecircSt_flg_ovrdval
  VTHC_sigSetTempZon1St_C_Inproc : FVT_lib/outp/OverrideAndLimit  SystemSampleTime=-1  VariantActivationTime=update diagram  Latency=0  AutoFrameSizeCalculation=off
      link override Signal_Limit/_maxval: Value=KOUTP_sigSetTempZon1St_C_maxval
      link override Signal_Limit/_minval: Value=KOUTP_sigSetTempZon1St_C_minval
      link override Signal_Override/_ovrdflg: Value=KOUTP_sigSetTempZon1St_C_ovrdflg
      link override Signal_Override/_ovrdval: Value=KOUTP_sigSetTempZon1St_C_ovrdval
  VTHC_sigSetTempZon2StM_C_Inproc : FVT_lib/outp/OverrideAndLimit  SystemSampleTime=-1  VariantActivationTime=update diagram  Latency=0  AutoFrameSizeCalculation=off
      link override Signal_Limit/_maxval: Value=KOUTP_sigSetTempZon2StM_C_maxval
      link override Signal_Limit/_minval: Value=KOUTP_sigSetTempZon2StM_C_minval
      link override Signal_Override/_ovrdflg: Value=KOUTP_sigSetTempZon2StM_C_ovrdflg
      link override Signal_Override/_ovrdval: Value=KOUTP_sigSetTempZon2StM_C_ovrdval
  VTHC_sigSetTempZon2St_C_Inproc : FVT_lib/outp/OverrideAndLimit  SystemSampleTime=-1  VariantActivationTime=update diagram  Latency=0  AutoFrameSizeCalculation=off
      link override Signal_Limit/_maxval: Value=KOUTP_sigSetTempZon2St_C_maxval
      link override Signal_Limit/_minval: Value=KOUTP_sigSetTempZon2St_C_minval
      link override Signal_Override/_ovrdflg: Value=KOUTP_sigSetTempZon2St_C_ovrdflg
      link override Signal_Override/_ovrdval: Value=KOUTP_sigSetTempZon2St_C_ovrdval
  VTHC_sigWindDirZon1St_enum_Inproc : FVT_lib/outp/OverrideAndLimit  SystemSampleTime=-1  VariantActivationTime=update diagram  Latency=0  AutoFrameSizeCalculation=off
      link override Signal_Limit/_maxval: Value=KOUTP_sigWindDirZon1St_enum_maxval
      link override Signal_Limit/_minval: Value=KOUTP_sigWindDirZon1St_enum_minval
      link override Signal_Override/_ovrdflg: Value=KOUTP_sigWindDirZon1St_enum_ovrdflg
      link override Signal_Override/_ovrdval: Value=KOUTP_sigWindDirZon1St_enum_ovrdval
  VTPM_ALFin_flg_Inproc : FVT_lib/outp/OverrideAndLimit  SystemSampleTime=-1  VariantActivationTime=update diagram  Latency=0  AutoFrameSizeCalculation=off
      link override Signal_Limit/_maxval: Value=KOUTP_ALFin_flg_maxval
      link override Signal_Limit/_minval: Value=KOUTP_ALFin_flg_minval
      link override Signal_Override/_ovrdflg: Value=KOUTP_ALFin_flg_ovrdflg
      link override Signal_Override/_ovrdval: Value=KOUTP_ALFin_flg_ovrdval
  VTPM_AutoLTips_enum_Inproc : FVT_lib/outp/OverrideAndLimit  SystemSampleTime=-1  VariantActivationTime=update diagram  Latency=0  AutoFrameSizeCalculation=off
      link override Signal_Limit/_maxval: Value=KOUTP_AutoLTips_enum_maxval
      link override Signal_Limit/_minval: Value=KOUTP_AutoLTips_enum_minval
      link override Signal_Override/_ovrdflg: Value=KOUTP_AutoLTips_enum_ovrdflg
      link override Signal_Override/_ovrdval: Value=KOUTP_AutoLTips_enum_ovrdval
  VTPM_CWheelTips_enum_Inproc : FVT_lib/outp/OverrideAndLimit  SystemSampleTime=-1  VariantActivationTime=update diagram  Latency=0  AutoFrameSizeCalculation=off
      link override Signal_Limit/_maxval: Value=KOUTP_CWheelTips_enum_maxval
      link override Signal_Limit/_minval: Value=KOUTP_CWheelTips_enum_minval
      link override Signal_Override/_ovrdflg: Value=KOUTP_CWheelTips_enum_ovrdflg
      link override Signal_Override/_ovrdval: Value=KOUTP_CWheelTips_enum_ovrdval
  VTPM_ChkStorge_flg_Inproc : FVT_lib/outp/OverrideAndLimit  SystemSampleTime=-1  VariantActivationTime=update diagram  Latency=0  AutoFrameSizeCalculation=off
      link override Signal_Limit/_maxval: Value=KOUTP_ChkStorge_flg_maxval
      link override Signal_Limit/_minval: Value=KOUTP_ChkStorge_flg_minval
      link override Signal_Override/_ovrdflg: Value=KOUTP_ChkStorge_flg_ovrdflg
      link override Signal_Override/_ovrdval: Value=KOUTP_ChkStorge_flg_ovrdval
  VTPM_Chkfin_flg_Inproc : FVT_lib/outp/OverrideAndLimit  SystemSampleTime=-1  VariantActivationTime=update diagram  Latency=0  AutoFrameSizeCalculation=off
      link override Signal_Limit/_maxval: Value=KOUTP_Chkfin_flg_maxval
      link override Signal_Limit/_minval: Value=KOUTP_Chkfin_flg_minval
      link override Signal_Override/_ovrdflg: Value=KOUTP_Chkfin_flg_ovrdflg
      link override Signal_Override/_ovrdval: Value=KOUTP_Chkfin_flg_ovrdval
  VTPM_FAT_flg_Inproc : FVT_lib/outp/OverrideAndLimit  SystemSampleTime=-1  VariantActivationTime=update diagram  Latency=0  AutoFrameSizeCalculation=off
      link override Signal_Limit/_maxval: Value=KOUTP_FAT_flg_maxval
      link override Signal_Limit/_minval: Value=KOUTP_FAT_flg_minval
      link override Signal_Override/_ovrdflg: Value=KOUTP_FAT_flg_ovrdflg
      link override Signal_Override/_ovrdval: Value=KOUTP_FAT_flg_ovrdval
  VTPM_FlashIDvalid_enum_Inproc : FVT_lib/outp/OverrideAndLimit  SystemSampleTime=-1  VariantActivationTime=update diagram  Latency=0  AutoFrameSizeCalculation=off
      link override Signal_Limit/_maxval: Value=KOUTP_FlashIDvalid_enum_maxval
      link override Signal_Limit/_minval: Value=KOUTP_FlashIDvalid_enum_minval
      link override Signal_Override/_ovrdflg: Value=KOUTP_FlashIDvalid_enum_ovrdflg
      link override Signal_Override/_ovrdval: Value=KOUTP_FlashIDvalid_enum_ovrdval
  VTPM_FlashS1ID_raw_Inproc : FVT_lib/outp/OverrideAndLimit  SystemSampleTime=-1  VariantActivationTime=update diagram  Latency=0  AutoFrameSizeCalculation=off
      link override Signal_Limit/_maxval: Value=KOUTP_FlashS1ID_raw_maxval
      link override Signal_Limit/_minval: Value=KOUTP_FlashS1ID_raw_minval
      link override Signal_Override/_ovrdflg: Value=KOUTP_FlashS1ID_raw_ovrdflg
      link override Signal_Override/_ovrdval: Value=KOUTP_FlashS1ID_raw_ovrdval
  VTPM_FlashS2ID_raw_Inproc : FVT_lib/outp/OverrideAndLimit  SystemSampleTime=-1  VariantActivationTime=update diagram  Latency=0  AutoFrameSizeCalculation=off
      link override Signal_Limit/_maxval: Value=KOUTP_FlashS2ID_raw_maxval
      link override Signal_Limit/_minval: Value=KOUTP_FlashS2ID_raw_minval
      link override Signal_Override/_ovrdflg: Value=KOUTP_FlashS2ID_raw_ovrdflg
      link override Signal_Override/_ovrdval: Value=KOUTP_FlashS2ID_raw_ovrdval
  VTPM_FlashS3ID_raw_Inproc : FVT_lib/outp/OverrideAndLimit  SystemSampleTime=-1  VariantActivationTime=update diagram  Latency=0  AutoFrameSizeCalculation=off
      link override Signal_Limit/_maxval: Value=KOUTP_FlashS3ID_raw_maxval
      link override Signal_Limit/_minval: Value=KOUTP_FlashS3ID_raw_minval
      link override Signal_Override/_ovrdflg: Value=KOUTP_FlashS3ID_raw_ovrdflg
      link override Signal_Override/_ovrdval: Value=KOUTP_FlashS3ID_raw_ovrdval
  VTPM_FlashS4ID_raw_Inproc : FVT_lib/outp/OverrideAndLimit  SystemSampleTime=-1  VariantActivationTime=update diagram  Latency=0  AutoFrameSizeCalculation=off
      link override Signal_Limit/_maxval: Value=KOUTP_FlashS4ID_raw_maxval
      link override Signal_Limit/_minval: Value=KOUTP_FlashS4ID_raw_minval
      link override Signal_Override/_ovrdflg: Value=KOUTP_FlashS4ID_raw_ovrdflg
      link override Signal_Override/_ovrdval: Value=KOUTP_FlashS4ID_raw_ovrdval
  VTPM_Flashchkdatavalid_enum_Inproc : FVT_lib/outp/OverrideAndLimit  SystemSampleTime=-1  VariantActivationTime=update diagram  Latency=0  AutoFrameSizeCalculation=off
      link override Signal_Limit/_maxval: Value=KOUTP_Flashchkdatavalid_enum_maxval
      link override Signal_Limit/_minval: Value=KOUTP_Flashchkdatavalid_enum_minval
      link override Signal_Override/_ovrdflg: Value=KOUTP_Flashchkdatavalid_enum_ovrdflg
      link override Signal_Override/_ovrdval: Value=KOUTP_Flashchkdatavalid_enum_ovrdval
  VTPM_Flashdatavalid_enum_Inproc : FVT_lib/outp/OverrideAndLimit  SystemSampleTime=-1  VariantActivationTime=update diagram  Latency=0  AutoFrameSizeCalculation=off
      link override Signal_Limit/_maxval: Value=KOUTP_Flashdatavalid_enum_maxval
      link override Signal_Limit/_minval: Value=KOUTP_Flashdatavalid_enum_minval
      link override Signal_Override/_ovrdflg: Value=KOUTP_Flashdatavalid_enum_ovrdflg
      link override Signal_Override/_ovrdval: Value=KOUTP_Flashdatavalid_enum_ovrdval
  VTPM_ID1messageALTU_raw8_Inproc : FVT_lib/outp/OverrideAndLimit  SystemSampleTime=-1  VariantActivationTime=update diagram  Latency=0  AutoFrameSizeCalculation=off
      link override Signal_Limit/_maxval: Value=KOUTP_ID1messageALTU_raw8_maxval
      link override Signal_Limit/_minval: Value=KOUTP_ID1messageALTU_raw8_minval
      link override Signal_Override/_ovrdflg: Value=KOUTP_ID1messageALTU_raw8_ovrdflg
      link override Signal_Override/_ovrdval: Value=KOUTP_ID1messageALTU_raw8_ovrdval
  VTPM_ID2messageALTU_raw8_Inproc : FVT_lib/outp/OverrideAndLimit  SystemSampleTime=-1  VariantActivationTime=update diagram  Latency=0  AutoFrameSizeCalculation=off
      link override Signal_Limit/_maxval: Value=KOUTP_ID2messageALTU_raw8_maxval
      link override Signal_Limit/_minval: Value=KOUTP_ID2messageALTU_raw8_minval
      link override Signal_Override/_ovrdflg: Value=KOUTP_ID2messageALTU_raw8_ovrdflg
      link override Signal_Override/_ovrdval: Value=KOUTP_ID2messageALTU_raw8_ovrdval
  VTPM_ID3messageALTU_raw8_Inproc : FVT_lib/outp/OverrideAndLimit  SystemSampleTime=-1  VariantActivationTime=update diagram  Latency=0  AutoFrameSizeCalculation=off
      link override Signal_Limit/_maxval: Value=KOUTP_ID3messageALTU_raw8_maxval
      link override Signal_Limit/_minval: Value=KOUTP_ID3messageALTU_raw8_minval
      link override Signal_Override/_ovrdflg: Value=KOUTP_ID3messageALTU_raw8_ovrdflg
      link override Signal_Override/_ovrdval: Value=KOUTP_ID3messageALTU_raw8_ovrdval
  VTPM_ID4messageALTU_raw8_Inproc : FVT_lib/outp/OverrideAndLimit  SystemSampleTime=-1  VariantActivationTime=update diagram  Latency=0  AutoFrameSizeCalculation=off
      link override Signal_Limit/_maxval: Value=KOUTP_ID4messageALTU_raw8_maxval
      link override Signal_Limit/_minval: Value=KOUTP_ID4messageALTU_raw8_minval
      link override Signal_Override/_ovrdflg: Value=KOUTP_ID4messageALTU_raw8_ovrdflg
      link override Signal_Override/_ovrdval: Value=KOUTP_ID4messageALTU_raw8_ovrdval
  VTPM_IDin_raw32_Inproc : FVT_lib/outp/OverrideAndLimit  SystemSampleTime=-1  VariantActivationTime=update diagram  Latency=0  AutoFrameSizeCalculation=off
      link override Signal_Limit/_maxval: Value=KOUTP_IDin_raw32_maxval
      link override Signal_Limit/_minval: Value=KOUTP_IDin_raw32_minval
      link override Signal_Override/_ovrdflg: Value=KOUTP_IDin_raw32_ovrdflg
      link override Signal_Override/_ovrdval: Value=KOUTP_IDin_raw32_ovrdval
  VTPM_LFBatWarn_flg_Inproc : FVT_lib/outp/OverrideAndLimit  SystemSampleTime=-1  VariantActivationTime=update diagram  Latency=0  AutoFrameSizeCalculation=off
      link override Signal_Limit/_maxval: Value=KOUTP_LFBatWarn_flg_maxval
      link override Signal_Limit/_minval: Value=KOUTP_LFBatWarn_flg_minval
      link override Signal_Override/_ovrdflg: Value=KOUTP_LFBatWarn_flg_ovrdflg
      link override Signal_Override/_ovrdval: Value=KOUTP_LFBatWarn_flg_ovrdval
  VTPM_LFP20_raw8_Inproc : FVT_lib/outp/OverrideAndLimit  SystemSampleTime=-1  VariantActivationTime=update diagram  Latency=0  AutoFrameSizeCalculation=off
      link override Signal_Limit/_maxval: Value=KOUTP_LFP20_raw8_maxval
      link override Signal_Limit/_minval: Value=KOUTP_LFP20_raw8_minval
      link override Signal_Override/_ovrdflg: Value=KOUTP_LFP20_raw8_ovrdflg
      link override Signal_Override/_ovrdval: Value=KOUTP_LFP20_raw8_ovrdval
  VTPM_LFPindi_enum_Inproc : FVT_lib/outp/OverrideAndLimit  SystemSampleTime=-1  VariantActivationTime=update diagram  Latency=0  AutoFrameSizeCalculation=off
      link override Signal_Limit/_maxval: Value=KOUTP_LFPindi_enum_maxval
      link override Signal_Limit/_minval: Value=KOUTP_LFPindi_enum_minval
      link override Signal_Override/_ovrdflg: Value=KOUTP_LFPindi_enum_ovrdflg
      link override Signal_Override/_ovrdval: Value=KOUTP_LFPindi_enum_ovrdval
  VTPM_LFPressIndi_enum_Inproc : FVT_lib/outp/OverrideAndLimit  SystemSampleTime=-1  VariantActivationTime=update diagram  Latency=0  AutoFrameSizeCalculation=off
      link override Signal_Limit/_maxval: Value=KOUTP_LFPressIndi_enum_maxval
      link override Signal_Limit/_minval: Value=KOUTP_LFPressIndi_enum_minval
      link override Signal_Override/_ovrdflg: Value=KOUTP_LFPressIndi_enum_ovrdflg
      link override Signal_Override/_ovrdval: Value=KOUTP_LFPressIndi_enum_ovrdval
  VTPM_LFSensorFail_flg_Inproc : FVT_lib/outp/OverrideAndLimit  SystemSampleTime=-1  VariantActivationTime=update diagram  Latency=0  AutoFrameSizeCalculation=off
      link override Signal_Limit/_maxval: Value=KOUTP_LFSensorFail_flg_maxval
      link override Signal_Limit/_minval: Value=KOUTP_LFSensorFail_flg_minval
      link override Signal_Override/_ovrdflg: Value=KOUTP_LFSensorFail_flg_ovrdflg
      link override Signal_Override/_ovrdval: Value=KOUTP_LFSensorFail_flg_ovrdval
  VTPM_LFSensorMode_flg_Inproc : FVT_lib/outp/OverrideAndLimit  SystemSampleTime=-1  VariantActivationTime=update diagram  Latency=0  AutoFrameSizeCalculation=off
      link override Signal_Limit/_maxval: Value=KOUTP_LFSensorMode_flg_maxval
      link override Signal_Limit/_minval: Value=KOUTP_LFSensorMode_flg_minval
      link override Signal_Override/_ovrdflg: Value=KOUTP_LFSensorMode_flg_ovrdflg
      link override Signal_Override/_ovrdval: Value=KOUTP_LFSensorMode_flg_ovrdval
  VTPM_LFWheelDebug_flg_Inproc : FVT_lib/outp/OverrideAndLimit  SystemSampleTime=-1  VariantActivationTime=update diagram  Latency=0  AutoFrameSizeCalculation=off
      link override Signal_Limit/_maxval: Value=KOUTP_LFWheelDebug_flg_maxval
      link override Signal_Limit/_minval: Value=KOUTP_LFWheelDebug_flg_minval
      link override Signal_Override/_ovrdflg: Value=KOUTP_LFWheelDebug_flg_ovrdflg
      link override Signal_Override/_ovrdval: Value=KOUTP_LFWheelDebug_flg_ovrdval
  VTPM_LFWheelPSW_raw8_Inproc : FVT_lib/outp/OverrideAndLimit  SystemSampleTime=-1  VariantActivationTime=update diagram  Latency=0  AutoFrameSizeCalculation=off
      link override Signal_Limit/_maxval: Value=KOUTP_LFWheelPSW_raw8_maxval
      link override Signal_Limit/_minval: Value=KOUTP_LFWheelPSW_raw8_minval
      link override Signal_Override/_ovrdflg: Value=KOUTP_LFWheelPSW_raw8_ovrdflg
      link override Signal_Override/_ovrdval: Value=KOUTP_LFWheelPSW_raw8_ovrdval
  VTPM_LFWheelPress_raw8_Inproc : FVT_lib/outp/OverrideAndLimit  SystemSampleTime=-1  VariantActivationTime=update diagram  Latency=0  AutoFrameSizeCalculation=off
      link override Signal_Limit/_maxval: Value=KOUTP_LFWheelPress_raw8_maxval
      link override Signal_Limit/_minval: Value=KOUTP_LFWheelPress_raw8_minval
      link override Signal_Override/_ovrdflg: Value=KOUTP_LFWheelPress_raw8_ovrdflg
      link override Signal_Override/_ovrdval: Value=KOUTP_LFWheelPress_raw8_ovrdval
  VTPM_LFWheelTemp_C_Inproc : FVT_lib/outp/OverrideAndLimit  SystemSampleTime=-1  VariantActivationTime=update diagram  Latency=0  AutoFrameSizeCalculation=off
      link override Signal_Limit/_maxval: Value=KOUTP_LFWheelTemp_C_maxval
      link override Signal_Limit/_minval: Value=KOUTP_LFWheelTemp_C_minval
      link override Signal_Override/_ovrdflg: Value=KOUTP_LFWheelTemp_C_ovrdflg
      link override Signal_Override/_ovrdval: Value=KOUTP_LFWheelTemp_C_ovrdval
  VTPM_LFWheelTmpIndi_flg_Inproc : FVT_lib/outp/OverrideAndLimit  SystemSampleTime=-1  VariantActivationTime=update diagram  Latency=0  AutoFrameSizeCalculation=off
      link override Signal_Limit/_maxval: Value=KOUTP_LFWheelTmpIndi_flg_maxval
      link override Signal_Limit/_minval: Value=KOUTP_LFWheelTmpIndi_flg_minval
      link override Signal_Override/_ovrdflg: Value=KOUTP_LFWheelTmpIndi_flg_ovrdflg
      link override Signal_Override/_ovrdval: Value=KOUTP_LFWheelTmpIndi_flg_ovrdval
  VTPM_LProgress_enum_Inproc : FVT_lib/outp/OverrideAndLimit  SystemSampleTime=-1  VariantActivationTime=update diagram  Latency=0  AutoFrameSizeCalculation=off
      link override Signal_Limit/_maxval: Value=KOUTP_LProgress_enum_maxval
      link override Signal_Limit/_minval: Value=KOUTP_LProgress_enum_minval
      link override Signal_Override/_ovrdflg: Value=KOUTP_LProgress_enum_ovrdflg
      link override Signal_Override/_ovrdval: Value=KOUTP_LProgress_enum_ovrdval
  VTPM_LRBatWarn_flg_Inproc : FVT_lib/outp/OverrideAndLimit  SystemSampleTime=-1  VariantActivationTime=update diagram  Latency=0  AutoFrameSizeCalculation=off
      link override Signal_Limit/_maxval: Value=KOUTP_LRBatWarn_flg_maxval
      link override Signal_Limit/_minval: Value=KOUTP_LRBatWarn_flg_minval
      link override Signal_Override/_ovrdflg: Value=KOUTP_LRBatWarn_flg_ovrdflg
      link override Signal_Override/_ovrdval: Value=KOUTP_LRBatWarn_flg_ovrdval
  VTPM_LRP20_raw8_Inproc : FVT_lib/outp/OverrideAndLimit  SystemSampleTime=-1  VariantActivationTime=update diagram  Latency=0  AutoFrameSizeCalculation=off
      link override Signal_Limit/_maxval: Value=KOUTP_LRP20_raw8_maxval
      link override Signal_Limit/_minval: Value=KOUTP_LRP20_raw8_minval
      link override Signal_Override/_ovrdflg: Value=KOUTP_LRP20_raw8_ovrdflg
      link override Signal_Override/_ovrdval: Value=KOUTP_LRP20_raw8_ovrdval
  VTPM_LRPindi_enum_Inproc : FVT_lib/outp/OverrideAndLimit  SystemSampleTime=-1  VariantActivationTime=update diagram  Latency=0  AutoFrameSizeCalculation=off
      link override Signal_Limit/_maxval: Value=KOUTP_LRPindi_enum_maxval
      link override Signal_Limit/_minval: Value=KOUTP_LRPindi_enum_minval
      link override Signal_Override/_ovrdflg: Value=KOUTP_LRPindi_enum_ovrdflg
      link override Signal_Override/_ovrdval: Value=KOUTP_LRPindi_enum_ovrdval
  VTPM_LRPressIndi_enum_Inproc : FVT_lib/outp/OverrideAndLimit  SystemSampleTime=-1  VariantActivationTime=update diagram  Latency=0  AutoFrameSizeCalculation=off
      link override Signal_Limit/_maxval: Value=KOUTP_LRPressIndi_enum_maxval
      link override Signal_Limit/_minval: Value=KOUTP_LRPressIndi_enum_minval
      link override Signal_Override/_ovrdflg: Value=KOUTP_LRPressIndi_enum_ovrdflg
      link override Signal_Override/_ovrdval: Value=KOUTP_LRPressIndi_enum_ovrdval
  VTPM_LRSensorFail_flg_Inproc : FVT_lib/outp/OverrideAndLimit  SystemSampleTime=-1  VariantActivationTime=update diagram  Latency=0  AutoFrameSizeCalculation=off
      link override Signal_Limit/_maxval: Value=KOUTP_LRSensorFail_flg_maxval
      link override Signal_Limit/_minval: Value=KOUTP_LRSensorFail_flg_minval
      link override Signal_Override/_ovrdflg: Value=KOUTP_LRSensorFail_flg_ovrdflg
      link override Signal_Override/_ovrdval: Value=KOUTP_LRSensorFail_flg_ovrdval
  VTPM_LRSensorMode_flg_Inproc : FVT_lib/outp/OverrideAndLimit  SystemSampleTime=-1  VariantActivationTime=update diagram  Latency=0  AutoFrameSizeCalculation=off
      link override Signal_Limit/_maxval: Value=KOUTP_LRSensorMode_flg_maxval
      link override Signal_Limit/_minval: Value=KOUTP_LRSensorMode_flg_minval
      link override Signal_Override/_ovrdflg: Value=KOUTP_LRSensorMode_flg_ovrdflg
      link override Signal_Override/_ovrdval: Value=KOUTP_LRSensorMode_flg_ovrdval
  VTPM_LRWheelDebug_flg_Inproc : FVT_lib/outp/OverrideAndLimit  SystemSampleTime=-1  VariantActivationTime=update diagram  Latency=0  AutoFrameSizeCalculation=off
      link override Signal_Limit/_maxval: Value=KOUTP_LRWheelDebug_flg_maxval
      link override Signal_Limit/_minval: Value=KOUTP_LRWheelDebug_flg_minval
      link override Signal_Override/_ovrdflg: Value=KOUTP_LRWheelDebug_flg_ovrdflg
      link override Signal_Override/_ovrdval: Value=KOUTP_LRWheelDebug_flg_ovrdval
  VTPM_LRWheelPSW_raw8_Inproc : FVT_lib/outp/OverrideAndLimit  SystemSampleTime=-1  VariantActivationTime=update diagram  Latency=0  AutoFrameSizeCalculation=off
      link override Signal_Limit/_maxval: Value=KOUTP_LRWheelPSW_raw8_maxval
      link override Signal_Limit/_minval: Value=KOUTP_LRWheelPSW_raw8_minval
      link override Signal_Override/_ovrdflg: Value=KOUTP_LRWheelPSW_raw8_ovrdflg
      link override Signal_Override/_ovrdval: Value=KOUTP_LRWheelPSW_raw8_ovrdval
  VTPM_LRWheelPress_raw8_Inproc : FVT_lib/outp/OverrideAndLimit  SystemSampleTime=-1  VariantActivationTime=update diagram  Latency=0  AutoFrameSizeCalculation=off
      link override Signal_Limit/_maxval: Value=KOUTP_LRWheelPress_raw8_maxval
      link override Signal_Limit/_minval: Value=KOUTP_LRWheelPress_raw8_minval
      link override Signal_Override/_ovrdflg: Value=KOUTP_LRWheelPress_raw8_ovrdflg
      link override Signal_Override/_ovrdval: Value=KOUTP_LRWheelPress_raw8_ovrdval
  VTPM_LRWheelTemp_C_Inproc : FVT_lib/outp/OverrideAndLimit  SystemSampleTime=-1  VariantActivationTime=update diagram  Latency=0  AutoFrameSizeCalculation=off
      link override Signal_Limit/_maxval: Value=KOUTP_LRWheelTemp_C_maxval
      link override Signal_Limit/_minval: Value=KOUTP_LRWheelTemp_C_minval
      link override Signal_Override/_ovrdflg: Value=KOUTP_LRWheelTemp_C_ovrdflg
      link override Signal_Override/_ovrdval: Value=KOUTP_LRWheelTemp_C_ovrdval
  VTPM_LRWheelTmpIndi_flg_Inproc : FVT_lib/outp/OverrideAndLimit  SystemSampleTime=-1  VariantActivationTime=update diagram  Latency=0  AutoFrameSizeCalculation=off
      link override Signal_Limit/_maxval: Value=KOUTP_LRWheelTmpIndi_flg_maxval
      link override Signal_Limit/_minval: Value=KOUTP_LRWheelTmpIndi_flg_minval
      link override Signal_Override/_ovrdflg: Value=KOUTP_LRWheelTmpIndi_flg_ovrdflg
      link override Signal_Override/_ovrdval: Value=KOUTP_LRWheelTmpIndi_flg_ovrdval
  VTPM_ModelVersionChksum_raw_Inproc : FVT_lib/outp/OverrideAndLimit  SystemSampleTime=-1  VariantActivationTime=update diagram  Latency=0  AutoFrameSizeCalculation=off
      link override Signal_Limit/_maxval: Value=KOUTP_ModelVersionChksum_raw_maxval
      link override Signal_Limit/_minval: Value=KOUTP_ModelVersionChksum_raw_minval
      link override Signal_Override/_ovrdflg: Value=KOUTP_ModelVersionChksum_raw_ovrdflg
      link override Signal_Override/_ovrdval: Value=KOUTP_ModelVersionChksum_raw_ovrdval
  VTPM_ModelVersion_raw_Inproc : FVT_lib/outp/OverrideAndLimit  SystemSampleTime=-1  VariantActivationTime=update diagram  Latency=0  AutoFrameSizeCalculation=off
      link override Signal_Limit/_maxval: Value=KOUTP_ModelVersion_raw_maxval
      link override Signal_Limit/_minval: Value=KOUTP_ModelVersion_raw_minval
      link override Signal_Override/_ovrdflg: Value=KOUTP_ModelVersion_raw_ovrdflg
      link override Signal_Override/_ovrdval: Value=KOUTP_ModelVersion_raw_ovrdval
  VTPM_Prepresstempvalid_enum_Inproc : FVT_lib/outp/OverrideAndLimit  SystemSampleTime=-1  VariantActivationTime=update diagram  Latency=0  AutoFrameSizeCalculation=off
      link override Signal_Limit/_maxval: Value=KOUTP_Prepresstempvalid_enum_maxval
      link override Signal_Limit/_minval: Value=KOUTP_Prepresstempvalid_enum_minval
      link override Signal_Override/_ovrdflg: Value=KOUTP_Prepresstempvalid_enum_ovrdflg
      link override Signal_Override/_ovrdval: Value=KOUTP_Prepresstempvalid_enum_ovrdval
  VTPM_RFBatWarn_flg_Inproc : FVT_lib/outp/OverrideAndLimit  SystemSampleTime=-1  VariantActivationTime=update diagram  Latency=0  AutoFrameSizeCalculation=off
      link override Signal_Limit/_maxval: Value=KOUTP_RFBatWarn_flg_maxval
      link override Signal_Limit/_minval: Value=KOUTP_RFBatWarn_flg_minval
      link override Signal_Override/_ovrdflg: Value=KOUTP_RFBatWarn_flg_ovrdflg
      link override Signal_Override/_ovrdval: Value=KOUTP_RFBatWarn_flg_ovrdval
  VTPM_RFP20_raw8_Inproc : FVT_lib/outp/OverrideAndLimit  SystemSampleTime=-1  VariantActivationTime=update diagram  Latency=0  AutoFrameSizeCalculation=off
      link override Signal_Limit/_maxval: Value=KOUTP_RFP20_raw8_maxval
      link override Signal_Limit/_minval: Value=KOUTP_RFP20_raw8_minval
      link override Signal_Override/_ovrdflg: Value=KOUTP_RFP20_raw8_ovrdflg
      link override Signal_Override/_ovrdval: Value=KOUTP_RFP20_raw8_ovrdval
  VTPM_RFPind_enum_Inproc : FVT_lib/outp/OverrideAndLimit  SystemSampleTime=-1  VariantActivationTime=update diagram  Latency=0  AutoFrameSizeCalculation=off
      link override Signal_Limit/_maxval: Value=KOUTP_RFPind_enum_maxval
      link override Signal_Limit/_minval: Value=KOUTP_RFPind_enum_minval
      link override Signal_Override/_ovrdflg: Value=KOUTP_RFPind_enum_ovrdflg
      link override Signal_Override/_ovrdval: Value=KOUTP_RFPind_enum_ovrdval
  VTPM_RFPressIndi_enum_Inproc : FVT_lib/outp/OverrideAndLimit  SystemSampleTime=-1  VariantActivationTime=update diagram  Latency=0  AutoFrameSizeCalculation=off
      link override Signal_Limit/_maxval: Value=KOUTP_RFPressIndi_enum_maxval
      link override Signal_Limit/_minval: Value=KOUTP_RFPressIndi_enum_minval
      link override Signal_Override/_ovrdflg: Value=KOUTP_RFPressIndi_enum_ovrdflg
      link override Signal_Override/_ovrdval: Value=KOUTP_RFPressIndi_enum_ovrdval
  VTPM_RFSensorFail_flg_Inproc : FVT_lib/outp/OverrideAndLimit  SystemSampleTime=-1  VariantActivationTime=update diagram  Latency=0  AutoFrameSizeCalculation=off
      link override Signal_Limit/_maxval: Value=KOUTP_RFSensorFail_flg_maxval
      link override Signal_Limit/_minval: Value=KOUTP_RFSensorFail_flg_minval
      link override Signal_Override/_ovrdflg: Value=KOUTP_RFSensorFail_flg_ovrdflg
      link override Signal_Override/_ovrdval: Value=KOUTP_RFSensorFail_flg_ovrdval
  VTPM_RFSensorMode_flg_Inproc : FVT_lib/outp/OverrideAndLimit  SystemSampleTime=-1  VariantActivationTime=update diagram  Latency=0  AutoFrameSizeCalculation=off
      link override Signal_Limit/_maxval: Value=KOUTP_RFSensorMode_flg_maxval
      link override Signal_Limit/_minval: Value=KOUTP_RFSensorMode_flg_minval
      link override Signal_Override/_ovrdflg: Value=KOUTP_RFSensorMode_flg_ovrdflg
      link override Signal_Override/_ovrdval: Value=KOUTP_RFSensorMode_flg_ovrdval
  VTPM_RFWheelDebug_flg_Inproc : FVT_lib/outp/OverrideAndLimit  SystemSampleTime=-1  VariantActivationTime=update diagram  Latency=0  AutoFrameSizeCalculation=off
      link override Signal_Limit/_maxval: Value=KOUTP_RFWheelDebug_flg_maxval
      link override Signal_Limit/_minval: Value=KOUTP_RFWheelDebug_flg_minval
      link override Signal_Override/_ovrdflg: Value=KOUTP_RFWheelDebug_flg_ovrdflg
      link override Signal_Override/_ovrdval: Value=KOUTP_RFWheelDebug_flg_ovrdval
  VTPM_RFWheelPSW_raw8_Inproc : FVT_lib/outp/OverrideAndLimit  SystemSampleTime=-1  VariantActivationTime=update diagram  Latency=0  AutoFrameSizeCalculation=off
      link override Signal_Limit/_maxval: Value=KOUTP_RFWheelPSW_raw8_maxval
      link override Signal_Limit/_minval: Value=KOUTP_RFWheelPSW_raw8_minval
      link override Signal_Override/_ovrdflg: Value=KOUTP_RFWheelPSW_raw8_ovrdflg
      link override Signal_Override/_ovrdval: Value=KOUTP_RFWheelPSW_raw8_ovrdval
  VTPM_RFWheelPress_raw8_Inproc : FVT_lib/outp/OverrideAndLimit  SystemSampleTime=-1  VariantActivationTime=update diagram  Latency=0  AutoFrameSizeCalculation=off
      link override Signal_Limit/_maxval: Value=KOUTP_RFWheelPress_raw8_maxval
      link override Signal_Limit/_minval: Value=KOUTP_RFWheelPress_raw8_minval
      link override Signal_Override/_ovrdflg: Value=KOUTP_RFWheelPress_raw8_ovrdflg
      link override Signal_Override/_ovrdval: Value=KOUTP_RFWheelPress_raw8_ovrdval
  VTPM_RFWheelTemp_C_Inproc : FVT_lib/outp/OverrideAndLimit  SystemSampleTime=-1  VariantActivationTime=update diagram  Latency=0  AutoFrameSizeCalculation=off
      link override Signal_Limit/_maxval: Value=KOUTP_RFWheelTemp_C_maxval
      link override Signal_Limit/_minval: Value=KOUTP_RFWheelTemp_C_minval
      link override Signal_Override/_ovrdflg: Value=KOUTP_RFWheelTemp_C_ovrdflg
      link override Signal_Override/_ovrdval: Value=KOUTP_RFWheelTemp_C_ovrdval
  VTPM_RFWheelTmpIndi_flg_Inproc : FVT_lib/outp/OverrideAndLimit  SystemSampleTime=-1  VariantActivationTime=update diagram  Latency=0  AutoFrameSizeCalculation=off
      link override Signal_Limit/_maxval: Value=KOUTP_RFWheelTmpIndi_flg_maxval
      link override Signal_Limit/_minval: Value=KOUTP_RFWheelTmpIndi_flg_minval
      link override Signal_Override/_ovrdflg: Value=KOUTP_RFWheelTmpIndi_flg_ovrdflg
      link override Signal_Override/_ovrdval: Value=KOUTP_RFWheelTmpIndi_flg_ovrdval
  VTPM_RRBatWarn_flg_Inproc : FVT_lib/outp/OverrideAndLimit  SystemSampleTime=-1  VariantActivationTime=update diagram  Latency=0  AutoFrameSizeCalculation=off
      link override Signal_Limit/_maxval: Value=KOUTP_RRBatWarn_flg_maxval
      link override Signal_Limit/_minval: Value=KOUTP_RRBatWarn_flg_minval
      link override Signal_Override/_ovrdflg: Value=KOUTP_RRBatWarn_flg_ovrdflg
      link override Signal_Override/_ovrdval: Value=KOUTP_RRBatWarn_flg_ovrdval
  VTPM_RRP20_raw8_Inproc : FVT_lib/outp/OverrideAndLimit  SystemSampleTime=-1  VariantActivationTime=update diagram  Latency=0  AutoFrameSizeCalculation=off
      link override Signal_Limit/_maxval: Value=KOUTP_RRP20_raw8_maxval
      link override Signal_Limit/_minval: Value=KOUTP_RRP20_raw8_minval
      link override Signal_Override/_ovrdflg: Value=KOUTP_RRP20_raw8_ovrdflg
      link override Signal_Override/_ovrdval: Value=KOUTP_RRP20_raw8_ovrdval
  VTPM_RRPindi_enum_Inproc : FVT_lib/outp/OverrideAndLimit  SystemSampleTime=-1  VariantActivationTime=update diagram  Latency=0  AutoFrameSizeCalculation=off
      link override Signal_Limit/_maxval: Value=KOUTP_RRPindi_enum_maxval
      link override Signal_Limit/_minval: Value=KOUTP_RRPindi_enum_minval
      link override Signal_Override/_ovrdflg: Value=KOUTP_RRPindi_enum_ovrdflg
      link override Signal_Override/_ovrdval: Value=KOUTP_RRPindi_enum_ovrdval
  VTPM_RRPressIndi_enum_Inproc : FVT_lib/outp/OverrideAndLimit  SystemSampleTime=-1  VariantActivationTime=update diagram  Latency=0  AutoFrameSizeCalculation=off
      link override Signal_Limit/_maxval: Value=KOUTP_RRPressIndi_enum_maxval
      link override Signal_Limit/_minval: Value=KOUTP_RRPressIndi_enum_minval
      link override Signal_Override/_ovrdflg: Value=KOUTP_RRPressIndi_enum_ovrdflg
      link override Signal_Override/_ovrdval: Value=KOUTP_RRPressIndi_enum_ovrdval
  VTPM_RRSensorFail_flg_Inproc : FVT_lib/outp/OverrideAndLimit  SystemSampleTime=-1  VariantActivationTime=update diagram  Latency=0  AutoFrameSizeCalculation=off
      link override Signal_Limit/_maxval: Value=KOUTP_RRSensorFail_flg_maxval
      link override Signal_Limit/_minval: Value=KOUTP_RRSensorFail_flg_minval
      link override Signal_Override/_ovrdflg: Value=KOUTP_RRSensorFail_flg_ovrdflg
      link override Signal_Override/_ovrdval: Value=KOUTP_RRSensorFail_flg_ovrdval
  VTPM_RRSensorMode_flg_Inproc : FVT_lib/outp/OverrideAndLimit  SystemSampleTime=-1  VariantActivationTime=update diagram  Latency=0  AutoFrameSizeCalculation=off
      link override Signal_Limit/_maxval: Value=KOUTP_RRSensorMode_flg_maxval
      link override Signal_Limit/_minval: Value=KOUTP_RRSensorMode_flg_minval
      link override Signal_Override/_ovrdflg: Value=KOUTP_RRSensorMode_flg_ovrdflg
      link override Signal_Override/_ovrdval: Value=KOUTP_RRSensorMode_flg_ovrdval
  VTPM_RRWheelDebug_flg_Inproc : FVT_lib/outp/OverrideAndLimit  SystemSampleTime=-1  VariantActivationTime=update diagram  Latency=0  AutoFrameSizeCalculation=off
      link override Signal_Limit/_maxval: Value=KOUTP_RRWheelDebug_flg_maxval
      link override Signal_Limit/_minval: Value=KOUTP_RRWheelDebug_flg_minval
      link override Signal_Override/_ovrdflg: Value=KOUTP_RRWheelDebug_flg_ovrdflg
      link override Signal_Override/_ovrdval: Value=KOUTP_RRWheelDebug_flg_ovrdval
  VTPM_RRWheelPSW_raw8_Inproc : FVT_lib/outp/OverrideAndLimit  SystemSampleTime=-1  VariantActivationTime=update diagram  Latency=0  AutoFrameSizeCalculation=off
      link override Signal_Limit/_maxval: Value=KOUTP_RRWheelPSW_raw8_maxval
      link override Signal_Limit/_minval: Value=KOUTP_RRWheelPSW_raw8_minval
      link override Signal_Override/_ovrdflg: Value=KOUTP_RRWheelPSW_raw8_ovrdflg
      link override Signal_Override/_ovrdval: Value=KOUTP_RRWheelPSW_raw8_ovrdval
  VTPM_RRWheelPress_raw8_Inproc : FVT_lib/outp/OverrideAndLimit  SystemSampleTime=-1  VariantActivationTime=update diagram  Latency=0  AutoFrameSizeCalculation=off
      link override Signal_Limit/_maxval: Value=KOUTP_RRWheelPress_raw8_maxval
      link override Signal_Limit/_minval: Value=KOUTP_RRWheelPress_raw8_minval
      link override Signal_Override/_ovrdflg: Value=KOUTP_RRWheelPress_raw8_ovrdflg
      link override Signal_Override/_ovrdval: Value=KOUTP_RRWheelPress_raw8_ovrdval
  VTPM_RRWheelTemp_C_Inproc : FVT_lib/outp/OverrideAndLimit  SystemSampleTime=-1  VariantActivationTime=update diagram  Latency=0  AutoFrameSizeCalculation=off
      link override Signal_Limit/_maxval: Value=KOUTP_RRWheelTemp_C_maxval
      link override Signal_Limit/_minval: Value=KOUTP_RRWheelTemp_C_minval
      link override Signal_Override/_ovrdflg: Value=KOUTP_RRWheelTemp_C_ovrdflg
      link override Signal_Override/_ovrdval: Value=KOUTP_RRWheelTemp_C_ovrdval
  VTPM_RRWheelTmpIndi_flg_Inproc : FVT_lib/outp/OverrideAndLimit  SystemSampleTime=-1  VariantActivationTime=update diagram  Latency=0  AutoFrameSizeCalculation=off
      link override Signal_Limit/_maxval: Value=KOUTP_RRWheelTmpIndi_flg_maxval
      link override Signal_Limit/_minval: Value=KOUTP_RRWheelTmpIndi_flg_minval
      link override Signal_Override/_ovrdflg: Value=KOUTP_RRWheelTmpIndi_flg_ovrdflg
      link override Signal_Override/_ovrdval: Value=KOUTP_RRWheelTmpIndi_flg_ovrdval
  VTPM_S1ID_raw32_Inproc : FVT_lib/outp/OverrideAndLimit  SystemSampleTime=-1  VariantActivationTime=update diagram  Latency=0  AutoFrameSizeCalculation=off
      link override Signal_Limit/_maxval: Value=KOUTP_S1ID_raw32_maxval
      link override Signal_Limit/_minval: Value=KOUTP_S1ID_raw32_minval
      link override Signal_Override/_ovrdflg: Value=KOUTP_S1ID_raw32_ovrdflg
      link override Signal_Override/_ovrdval: Value=KOUTP_S1ID_raw32_ovrdval
  VTPM_S1L_enum_Inproc : FVT_lib/outp/OverrideAndLimit  SystemSampleTime=-1  VariantActivationTime=update diagram  Latency=0  AutoFrameSizeCalculation=off
      link override Signal_Limit/_maxval: Value=KOUTP_S1L_enum_maxval
      link override Signal_Limit/_minval: Value=KOUTP_S1L_enum_minval
      link override Signal_Override/_ovrdflg: Value=KOUTP_S1L_enum_ovrdflg
      link override Signal_Override/_ovrdval: Value=KOUTP_S1L_enum_ovrdval
  VTPM_S1WheelDebugALTU_pct_Inproc : FVT_lib/outp/OverrideAndLimit  SystemSampleTime=-1  VariantActivationTime=update diagram  Latency=0  AutoFrameSizeCalculation=off
      link override Signal_Limit/_maxval: Value=KOUTP_S1WheelDebugALTU_pct_maxval
      link override Signal_Limit/_minval: Value=KOUTP_S1WheelDebugALTU_pct_minval
      link override Signal_Override/_ovrdflg: Value=KOUTP_S1WheelDebugALTU_pct_ovrdflg
      link override Signal_Override/_ovrdval: Value=KOUTP_S1WheelDebugALTU_pct_ovrdval
  VTPM_S2ID_raw32_Inproc : FVT_lib/outp/OverrideAndLimit  SystemSampleTime=-1  VariantActivationTime=update diagram  Latency=0  AutoFrameSizeCalculation=off
      link override Signal_Limit/_maxval: Value=KOUTP_S2ID_raw32_maxval
      link override Signal_Limit/_minval: Value=KOUTP_S2ID_raw32_minval
      link override Signal_Override/_ovrdflg: Value=KOUTP_S2ID_raw32_ovrdflg
      link override Signal_Override/_ovrdval: Value=KOUTP_S2ID_raw32_ovrdval
  VTPM_S2L_enum_Inproc : FVT_lib/outp/OverrideAndLimit  SystemSampleTime=-1  VariantActivationTime=update diagram  Latency=0  AutoFrameSizeCalculation=off
      link override Signal_Limit/_maxval: Value=KOUTP_S2L_enum_maxval
      link override Signal_Limit/_minval: Value=KOUTP_S2L_enum_minval
      link override Signal_Override/_ovrdflg: Value=KOUTP_S2L_enum_ovrdflg
      link override Signal_Override/_ovrdval: Value=KOUTP_S2L_enum_ovrdval
  VTPM_S2WheelDebugALTU_pct_Inproc : FVT_lib/outp/OverrideAndLimit  SystemSampleTime=-1  VariantActivationTime=update diagram  Latency=0  AutoFrameSizeCalculation=off
      link override Signal_Limit/_maxval: Value=KOUTP_S2WheelDebugALTU_pct_maxval
      link override Signal_Limit/_minval: Value=KOUTP_S2WheelDebugALTU_pct_minval
      link override Signal_Override/_ovrdflg: Value=KOUTP_S2WheelDebugALTU_pct_ovrdflg
      link override Signal_Override/_ovrdval: Value=KOUTP_S2WheelDebugALTU_pct_ovrdval
  VTPM_S3ID_raw32_Inproc : FVT_lib/outp/OverrideAndLimit  SystemSampleTime=-1  VariantActivationTime=update diagram  Latency=0  AutoFrameSizeCalculation=off
      link override Signal_Limit/_maxval: Value=KOUTP_S3ID_raw32_maxval
      link override Signal_Limit/_minval: Value=KOUTP_S3ID_raw32_minval
      link override Signal_Override/_ovrdflg: Value=KOUTP_S3ID_raw32_ovrdflg
      link override Signal_Override/_ovrdval: Value=KOUTP_S3ID_raw32_ovrdval
  VTPM_S3L_enum_Inproc : FVT_lib/outp/OverrideAndLimit  SystemSampleTime=-1  VariantActivationTime=update diagram  Latency=0  AutoFrameSizeCalculation=off
      link override Signal_Limit/_maxval: Value=KOUTP_S3L_enum_maxval
      link override Signal_Limit/_minval: Value=KOUTP_S3L_enum_minval
      link override Signal_Override/_ovrdflg: Value=KOUTP_S3L_enum_ovrdflg
      link override Signal_Override/_ovrdval: Value=KOUTP_S3L_enum_ovrdval
  VTPM_S3WheelDebugALTU_pct_Inproc : FVT_lib/outp/OverrideAndLimit  SystemSampleTime=-1  VariantActivationTime=update diagram  Latency=0  AutoFrameSizeCalculation=off
      link override Signal_Limit/_maxval: Value=KOUTP_S3WheelDebugALTU_pct_maxval
      link override Signal_Limit/_minval: Value=KOUTP_S3WheelDebugALTU_pct_minval
      link override Signal_Override/_ovrdflg: Value=KOUTP_S3WheelDebugALTU_pct_ovrdflg
      link override Signal_Override/_ovrdval: Value=KOUTP_S3WheelDebugALTU_pct_ovrdval
  VTPM_S4ID_raw32_Inproc : FVT_lib/outp/OverrideAndLimit  SystemSampleTime=-1  VariantActivationTime=update diagram  Latency=0  AutoFrameSizeCalculation=off
      link override Signal_Limit/_maxval: Value=KOUTP_S4ID_raw32_maxval
      link override Signal_Limit/_minval: Value=KOUTP_S4ID_raw32_minval
      link override Signal_Override/_ovrdflg: Value=KOUTP_S4ID_raw32_ovrdflg
      link override Signal_Override/_ovrdval: Value=KOUTP_S4ID_raw32_ovrdval
  VTPM_S4L_enum_Inproc : FVT_lib/outp/OverrideAndLimit  SystemSampleTime=-1  VariantActivationTime=update diagram  Latency=0  AutoFrameSizeCalculation=off
      link override Signal_Limit/_maxval: Value=KOUTP_S4L_enum_maxval
      link override Signal_Limit/_minval: Value=KOUTP_S4L_enum_minval
      link override Signal_Override/_ovrdflg: Value=KOUTP_S4L_enum_ovrdflg
      link override Signal_Override/_ovrdval: Value=KOUTP_S4L_enum_ovrdval
  VTPM_S4WheelDebugALTU_pct_Inproc : FVT_lib/outp/OverrideAndLimit  SystemSampleTime=-1  VariantActivationTime=update diagram  Latency=0  AutoFrameSizeCalculation=off
      link override Signal_Limit/_maxval: Value=KOUTP_S4WheelDebugALTU_pct_maxval
      link override Signal_Limit/_minval: Value=KOUTP_S4WheelDebugALTU_pct_minval
      link override Signal_Override/_ovrdflg: Value=KOUTP_S4WheelDebugALTU_pct_ovrdflg
      link override Signal_Override/_ovrdval: Value=KOUTP_S4WheelDebugALTU_pct_ovrdval
  VTPM_SetIDLoc_flg_Inproc : FVT_lib/outp/OverrideAndLimit  SystemSampleTime=-1  VariantActivationTime=update diagram  Latency=0  AutoFrameSizeCalculation=off
      link override Signal_Limit/_maxval: Value=KOUTP_SetIDLoc_flg_maxval
      link override Signal_Limit/_minval: Value=KOUTP_SetIDLoc_flg_minval
      link override Signal_Override/_ovrdflg: Value=KOUTP_SetIDLoc_flg_ovrdflg
      link override Signal_Override/_ovrdval: Value=KOUTP_SetIDLoc_flg_ovrdval
  VTPM_TPMSCaliButtAllow_flg_Inproc : FVT_lib/outp/OverrideAndLimit  SystemSampleTime=-1  VariantActivationTime=update diagram  Latency=0  AutoFrameSizeCalculation=off
      link override Signal_Limit/_maxval: Value=KOUTP_TPMSCaliButtAllow_flg_maxval
      link override Signal_Limit/_minval: Value=KOUTP_TPMSCaliButtAllow_flg_minval
      link override Signal_Override/_ovrdflg: Value=KOUTP_TPMSCaliButtAllow_flg_ovrdflg
      link override Signal_Override/_ovrdval: Value=KOUTP_TPMSCaliButtAllow_flg_ovrdval
  VTPM_TPMSResButtAllow_flg_Inproc : FVT_lib/outp/OverrideAndLimit  SystemSampleTime=-1  VariantActivationTime=update diagram  Latency=0  AutoFrameSizeCalculation=off
      link override Signal_Limit/_maxval: Value=KOUTP_TPMSResButtAllow_flg_maxval
      link override Signal_Limit/_minval: Value=KOUTP_TPMSResButtAllow_flg_minval
      link override Signal_Override/_ovrdflg: Value=KOUTP_TPMSResButtAllow_flg_ovrdflg
      link override Signal_Override/_ovrdval: Value=KOUTP_TPMSResButtAllow_flg_ovrdval
  VTPM_TPMSResButt_flg_Inproc : FVT_lib/outp/OverrideAndLimit  SystemSampleTime=-1  VariantActivationTime=update diagram  Latency=0  AutoFrameSizeCalculation=off
      link override Signal_Limit/_maxval: Value=KOUTP_TPMSResButt_flg_maxval
      link override Signal_Limit/_minval: Value=KOUTP_TPMSResButt_flg_minval
      link override Signal_Override/_ovrdflg: Value=KOUTP_TPMSResButt_flg_ovrdflg
      link override Signal_Override/_ovrdval: Value=KOUTP_TPMSResButt_flg_ovrdval
  VTPM_TPMSSensorIDRegStart_flg_Inproc : FVT_lib/outp/OverrideAndLimit  SystemSampleTime=-1  VariantActivationTime=update diagram  Latency=0  AutoFrameSizeCalculation=off
      link override Signal_Limit/_maxval: Value=KOUTP_TPMSSensorIDRegStart_flg_maxval
      link override Signal_Limit/_minval: Value=KOUTP_TPMSSensorIDRegStart_flg_minval
      link override Signal_Override/_ovrdflg: Value=KOUTP_TPMSSensorIDRegStart_flg_ovrdflg
      link override Signal_Override/_ovrdval: Value=KOUTP_TPMSSensorIDRegStart_flg_ovrdval
  VTPM_TPMSStorge_flg_Inproc : FVT_lib/outp/OverrideAndLimit  SystemSampleTime=-1  VariantActivationTime=update diagram  Latency=0  AutoFrameSizeCalculation=off
      link override Signal_Limit/_maxval: Value=KOUTP_TPMSStorge_flg_maxval
      link override Signal_Limit/_minval: Value=KOUTP_TPMSStorge_flg_minval
      link override Signal_Override/_ovrdflg: Value=KOUTP_TPMSStorge_flg_ovrdflg
      link override Signal_Override/_ovrdval: Value=KOUTP_TPMSStorge_flg_ovrdval
  VTPM_TPMSTLCmd_flg_Inproc : FVT_lib/outp/OverrideAndLimit  SystemSampleTime=-1  VariantActivationTime=update diagram  Latency=0  AutoFrameSizeCalculation=off
      link override Signal_Limit/_maxval: Value=KOUTP_TPMSTLCmd_flg_maxval
      link override Signal_Limit/_minval: Value=KOUTP_TPMSTLCmd_flg_minval
      link override Signal_Override/_ovrdflg: Value=KOUTP_TPMSTLCmd_flg_ovrdflg
      link override Signal_Override/_ovrdval: Value=KOUTP_TPMSTLCmd_flg_ovrdval
  VTPM_TPMSWarnIndi_enum_Inproc : FVT_lib/outp/OverrideAndLimit  SystemSampleTime=-1  VariantActivationTime=update diagram  Latency=0  AutoFrameSizeCalculation=off
      link override Signal_Limit/_maxval: Value=KOUTP_TPMSWarnIndi_enum_maxval
      link override Signal_Limit/_minval: Value=KOUTP_TPMSWarnIndi_enum_minval
      link override Signal_Override/_ovrdflg: Value=KOUTP_TPMSWarnIndi_enum_ovrdflg
      link override Signal_Override/_ovrdval: Value=KOUTP_TPMSWarnIndi_enum_ovrdval
  VTPM_WriteChkLFID_raw_Inproc : FVT_lib/outp/OverrideAndLimit  SystemSampleTime=-1  VariantActivationTime=update diagram  Latency=0  AutoFrameSizeCalculation=off
      link override Signal_Limit/_maxval: Value=KOUTP_WriteChkLFID_raw_maxval
      link override Signal_Limit/_minval: Value=KOUTP_WriteChkLFID_raw_minval
      link override Signal_Override/_ovrdflg: Value=KOUTP_WriteChkLFID_raw_ovrdflg
      link override Signal_Override/_ovrdval: Value=KOUTP_WriteChkLFID_raw_ovrdval
  VTPM_WriteChkLRID_raw_Inproc : FVT_lib/outp/OverrideAndLimit  SystemSampleTime=-1  VariantActivationTime=update diagram  Latency=0  AutoFrameSizeCalculation=off
      link override Signal_Limit/_maxval: Value=KOUTP_WriteChkLRID_raw_maxval
      link override Signal_Limit/_minval: Value=KOUTP_WriteChkLRID_raw_minval
      link override Signal_Override/_ovrdflg: Value=KOUTP_WriteChkLRID_raw_ovrdflg
      link override Signal_Override/_ovrdval: Value=KOUTP_WriteChkLRID_raw_ovrdval
  VTPM_WriteChkRFID_raw_Inproc : FVT_lib/outp/OverrideAndLimit  SystemSampleTime=-1  VariantActivationTime=update diagram  Latency=0  AutoFrameSizeCalculation=off
      link override Signal_Limit/_maxval: Value=KOUTP_WriteChkRFID_raw_maxval
      link override Signal_Limit/_minval: Value=KOUTP_WriteChkRFID_raw_minval
      link override Signal_Override/_ovrdflg: Value=KOUTP_WriteChkRFID_raw_ovrdflg
      link override Signal_Override/_ovrdval: Value=KOUTP_WriteChkRFID_raw_ovrdval
  VTPM_WriteChkRRID_raw_Inproc : FVT_lib/outp/OverrideAndLimit  SystemSampleTime=-1  VariantActivationTime=update diagram  Latency=0  AutoFrameSizeCalculation=off
      link override Signal_Limit/_maxval: Value=KOUTP_WriteChkRRID_raw_maxval
      link override Signal_Limit/_minval: Value=KOUTP_WriteChkRRID_raw_minval
      link override Signal_Override/_ovrdflg: Value=KOUTP_WriteChkRRID_raw_ovrdflg
      link override Signal_Override/_ovrdval: Value=KOUTP_WriteChkRRID_raw_ovrdval
  VTPM_WriteChkfinLFID_raw_Inproc : FVT_lib/outp/OverrideAndLimit  SystemSampleTime=-1  VariantActivationTime=update diagram  Latency=0  AutoFrameSizeCalculation=off
      link override Signal_Limit/_maxval: Value=KOUTP_WriteChkfinLFID_raw_maxval
      link override Signal_Limit/_minval: Value=KOUTP_WriteChkfinLFID_raw_minval
      link override Signal_Override/_ovrdflg: Value=KOUTP_WriteChkfinLFID_raw_ovrdflg
      link override Signal_Override/_ovrdval: Value=KOUTP_WriteChkfinLFID_raw_ovrdval
  VTPM_WriteChkfinLRID_raw_Inproc : FVT_lib/outp/OverrideAndLimit  SystemSampleTime=-1  VariantActivationTime=update diagram  Latency=0  AutoFrameSizeCalculation=off
      link override Signal_Limit/_maxval: Value=KOUTP_WriteChkfinLRID_raw_maxval
      link override Signal_Limit/_minval: Value=KOUTP_WriteChkfinLRID_raw_minval
      link override Signal_Override/_ovrdflg: Value=KOUTP_WriteChkfinLRID_raw_ovrdflg
      link override Signal_Override/_ovrdval: Value=KOUTP_WriteChkfinLRID_raw_ovrdval
  VTPM_WriteChkfinRFID_raw_Inproc : FVT_lib/outp/OverrideAndLimit  SystemSampleTime=-1  VariantActivationTime=update diagram  Latency=0  AutoFrameSizeCalculation=off
      link override Signal_Limit/_maxval: Value=KOUTP_WriteChkfinRFID_raw_maxval
      link override Signal_Limit/_minval: Value=KOUTP_WriteChkfinRFID_raw_minval
      link override Signal_Override/_ovrdflg: Value=KOUTP_WriteChkfinRFID_raw_ovrdflg
      link override Signal_Override/_ovrdval: Value=KOUTP_WriteChkfinRFID_raw_ovrdval
  VTPM_WriteChkfinRRID_raw_Inproc : FVT_lib/outp/OverrideAndLimit  SystemSampleTime=-1  VariantActivationTime=update diagram  Latency=0  AutoFrameSizeCalculation=off
      link override Signal_Limit/_maxval: Value=KOUTP_WriteChkfinRRID_raw_maxval
      link override Signal_Limit/_minval: Value=KOUTP_WriteChkfinRRID_raw_minval
      link override Signal_Override/_ovrdflg: Value=KOUTP_WriteChkfinRRID_raw_ovrdflg
      link override Signal_Override/_ovrdval: Value=KOUTP_WriteChkfinRRID_raw_ovrdval
  VTPM_WritingCnt_enum_Inproc : FVT_lib/outp/OverrideAndLimit  SystemSampleTime=-1  VariantActivationTime=update diagram  Latency=0  AutoFrameSizeCalculation=off
      link override Signal_Limit/_maxval: Value=KOUTP_WritingCnt_enum_maxval
      link override Signal_Limit/_minval: Value=KOUTP_WritingCnt_enum_minval
      link override Signal_Override/_ovrdflg: Value=KOUTP_WritingCnt_enum_ovrdflg
      link override Signal_Override/_ovrdval: Value=KOUTP_WritingCnt_enum_ovrdval
  VTPM_unlearnSfailvalid_enum_Inproc : FVT_lib/outp/OverrideAndLimit  SystemSampleTime=-1  VariantActivationTime=update diagram  Latency=0  AutoFrameSizeCalculation=off
      link override Signal_Limit/_maxval: Value=KOUTP_unlearnSfailvalid_enum_maxval
      link override Signal_Limit/_minval: Value=KOUTP_unlearnSfailvalid_enum_minval
      link override Signal_Override/_ovrdflg: Value=KOUTP_unlearnSfailvalid_enum_ovrdflg
      link override Signal_Override/_ovrdval: Value=KOUTP_unlearnSfailvalid_enum_ovrdval
  VTPM_unlearnSfali_flg_Inproc : FVT_lib/outp/OverrideAndLimit  SystemSampleTime=-1  VariantActivationTime=update diagram  Latency=0  AutoFrameSizeCalculation=off
      link override Signal_Limit/_maxval: Value=KOUTP_unlearnSfali_flg_maxval
      link override Signal_Limit/_minval: Value=KOUTP_unlearnSfali_flg_minval
      link override Signal_Override/_ovrdflg: Value=KOUTP_unlearnSfali_flg_ovrdflg
      link override Signal_Override/_ovrdval: Value=KOUTP_unlearnSfali_flg_ovrdval
  VTQD_ActParkRequest_flg_Inproc : FVT_lib/outp/OverrideAndLimit  SystemSampleTime=-1  VariantActivationTime=update diagram  Latency=0  AutoFrameSizeCalculation=off
      link override Signal_Limit/_maxval: Value=KOUTP_ActParkRequest_flg_maxval
      link override Signal_Limit/_minval: Value=KOUTP_ActParkRequest_flg_minval
      link override Signal_Override/_ovrdflg: Value=KOUTP_ActParkRequest_flg_ovrdflg
      link override Signal_Override/_ovrdval: Value=KOUTP_ActParkRequest_flg_ovrdval
  VTQD_CreepON_flg_Inproc : FVT_lib/outp/OverrideAndLimit  SystemSampleTime=-1  VariantActivationTime=update diagram  Latency=0  AutoFrameSizeCalculation=off
      link override Signal_Limit/_maxval: Value=KOUTP_CreepON_flg_maxval
      link override Signal_Limit/_minval: Value=KOUTP_CreepON_flg_minval
      link override Signal_Override/_ovrdflg: Value=KOUTP_CreepON_flg_ovrdflg
      link override Signal_Override/_ovrdval: Value=KOUTP_CreepON_flg_ovrdval
  VTQD_DriveProtEn_flg_Inproc : FVT_lib/outp/OverrideAndLimit  SystemSampleTime=-1  VariantActivationTime=update diagram  Latency=0  AutoFrameSizeCalculation=off
      link override Signal_Limit/_maxval: Value=KOUTP_DriveProtEn_flg_maxval
      link override Signal_Limit/_minval: Value=KOUTP_DriveProtEn_flg_minval
      link override Signal_Override/_ovrdflg: Value=KOUTP_DriveProtEn_flg_ovrdflg
      link override Signal_Override/_ovrdval: Value=KOUTP_DriveProtEn_flg_ovrdval
  VTQD_DriverWhlTqDemFr_Nm_Inproc : FVT_lib/outp/OverrideAndLimit  SystemSampleTime=-1  VariantActivationTime=update diagram  Latency=0  AutoFrameSizeCalculation=off
      link override Signal_Limit/_maxval: Value=KOUTP_DriverWhlTqDemFr_Nm_maxval
      link override Signal_Limit/_minval: Value=KOUTP_DriverWhlTqDemFr_Nm_minval
      link override Signal_Override/_ovrdflg: Value=KOUTP_DriverWhlTqDemFr_Nm_ovrdflg
      link override Signal_Override/_ovrdval: Value=KOUTP_DriverWhlTqDemFr_Nm_ovrdval
  VTQD_DriverWhlTqDemRr_Nm_Inproc : FVT_lib/outp/OverrideAndLimit  SystemSampleTime=-1  VariantActivationTime=update diagram  Latency=0  AutoFrameSizeCalculation=off
      link override Signal_Limit/_maxval: Value=KOUTP_DriverWhlTqDemRr_Nm_maxval
      link override Signal_Limit/_minval: Value=KOUTP_DriverWhlTqDemRr_Nm_minval
      link override Signal_Override/_ovrdflg: Value=KOUTP_DriverWhlTqDemRr_Nm_ovrdflg
      link override Signal_Override/_ovrdval: Value=KOUTP_DriverWhlTqDemRr_Nm_ovrdval
  VTQD_EVDriveMode_enum_Inproc : FVT_lib/outp/OverrideAndLimit  SystemSampleTime=-1  VariantActivationTime=update diagram  Latency=0  AutoFrameSizeCalculation=off
      link override Signal_Limit/_maxval: Value=KOUTP_EVDriveMode_enum_maxval
      link override Signal_Limit/_minval: Value=KOUTP_EVDriveMode_enum_minval
      link override Signal_Override/_ovrdflg: Value=KOUTP_EVDriveMode_enum_ovrdflg
      link override Signal_Override/_ovrdval: Value=KOUTP_EVDriveMode_enum_ovrdval
  VTQD_EquivAccPedalSWSta_flg_Inproc : FVT_lib/outp/OverrideAndLimit  SystemSampleTime=-1  VariantActivationTime=update diagram  Latency=0  AutoFrameSizeCalculation=off
      link override Signal_Limit/_maxval: Value=KOUTP_EquivAccPedalSWSta_flg_maxval
      link override Signal_Limit/_minval: Value=KOUTP_EquivAccPedalSWSta_flg_minval
      link override Signal_Override/_ovrdflg: Value=KOUTP_EquivAccPedalSWSta_flg_ovrdflg
      link override Signal_Override/_ovrdval: Value=KOUTP_EquivAccPedalSWSta_flg_ovrdval
  VTQD_FrActvDmpDisabReq_flg_Inproc : FVT_lib/outp/OverrideAndLimit  SystemSampleTime=-1  VariantActivationTime=update diagram  Latency=0  AutoFrameSizeCalculation=off
      link override Signal_Limit/_maxval: Value=KOUTP_FrActvDmpDisabReq_flg_maxval
      link override Signal_Limit/_minval: Value=KOUTP_FrActvDmpDisabReq_flg_minval
      link override Signal_Override/_ovrdflg: Value=KOUTP_FrActvDmpDisabReq_flg_ovrdflg
      link override Signal_Override/_ovrdval: Value=KOUTP_FrActvDmpDisabReq_flg_ovrdval
  VTQD_FrEDUActTq_Nm_Inproc : FVT_lib/outp/OverrideAndLimit  SystemSampleTime=-1  VariantActivationTime=update diagram  Latency=0  AutoFrameSizeCalculation=off
      link override Signal_Limit/_maxval: Value=KOUTP_FrEDUActTq_Nm_maxval
      link override Signal_Limit/_minval: Value=KOUTP_FrEDUActTq_Nm_minval
      link override Signal_Override/_ovrdflg: Value=KOUTP_FrEDUActTq_Nm_ovrdflg
      link override Signal_Override/_ovrdval: Value=KOUTP_FrEDUActTq_Nm_ovrdval
  VTQD_FrEDUAvailBrkRgnTqV_flg_Inproc : FVT_lib/outp/OverrideAndLimit  SystemSampleTime=-1  VariantActivationTime=update diagram  Latency=0  AutoFrameSizeCalculation=off
      link override Signal_Limit/_maxval: Value=KOUTP_FrEDUAvailBrkRgnTqV_flg_maxval
      link override Signal_Limit/_minval: Value=KOUTP_FrEDUAvailBrkRgnTqV_flg_minval
      link override Signal_Override/_ovrdflg: Value=KOUTP_FrEDUAvailBrkRgnTqV_flg_ovrdflg
      link override Signal_Override/_ovrdval: Value=KOUTP_FrEDUAvailBrkRgnTqV_flg_ovrdval
  VTQD_FrEDUAvailBrkRgnTq_Nm_Inproc : FVT_lib/outp/OverrideAndLimit  SystemSampleTime=-1  VariantActivationTime=update diagram  Latency=0  AutoFrameSizeCalculation=off
      link override Signal_Limit/_maxval: Value=KOUTP_FrEDUAvailBrkRgnTq_Nm_maxval
      link override Signal_Limit/_minval: Value=KOUTP_FrEDUAvailBrkRgnTq_Nm_minval
      link override Signal_Override/_ovrdflg: Value=KOUTP_FrEDUAvailBrkRgnTq_Nm_ovrdflg
      link override Signal_Override/_ovrdval: Value=KOUTP_FrEDUAvailBrkRgnTq_Nm_ovrdval
  VTQD_FrEDURolRgnTq_Nm_Inproc : FVT_lib/outp/OverrideAndLimit  SystemSampleTime=-1  VariantActivationTime=update diagram  Latency=0  AutoFrameSizeCalculation=off
      link override Signal_Limit/_maxval: Value=KOUTP_FrEDURolRgnTq_Nm_maxval
      link override Signal_Limit/_minval: Value=KOUTP_FrEDURolRgnTq_Nm_minval
      link override Signal_Override/_ovrdflg: Value=KOUTP_FrEDURolRgnTq_Nm_ovrdflg
      link override Signal_Override/_ovrdval: Value=KOUTP_FrEDURolRgnTq_Nm_ovrdval
  VTQD_FrEDUSpdValid_flg_Inproc : FVT_lib/outp/OverrideAndLimit  SystemSampleTime=-1  VariantActivationTime=update diagram  Latency=0  AutoFrameSizeCalculation=off
      link override Signal_Limit/_maxval: Value=KOUTP_FrEDUSpdValid_flg_maxval
      link override Signal_Limit/_minval: Value=KOUTP_FrEDUSpdValid_flg_minval
      link override Signal_Override/_ovrdflg: Value=KOUTP_FrEDUSpdValid_flg_ovrdflg
      link override Signal_Override/_ovrdval: Value=KOUTP_FrEDUSpdValid_flg_ovrdval
  VTQD_FrEDUSpd_rpm_Inproc : FVT_lib/outp/OverrideAndLimit  SystemSampleTime=-1  VariantActivationTime=update diagram  Latency=0  AutoFrameSizeCalculation=off
      link override Signal_Limit/_maxval: Value=KOUTP_FrEDUSpd_rpm_maxval
      link override Signal_Limit/_minval: Value=KOUTP_FrEDUSpd_rpm_minval
      link override Signal_Override/_ovrdflg: Value=KOUTP_FrEDUSpd_rpm_ovrdflg
      link override Signal_Override/_ovrdval: Value=KOUTP_FrEDUSpd_rpm_ovrdval
  VTQD_FrIdcMax_A_Inproc : FVT_lib/outp/OverrideAndLimit  SystemSampleTime=-1  VariantActivationTime=update diagram  Latency=0  AutoFrameSizeCalculation=off
      link override Signal_Limit/_maxval: Value=KOUTP_FrIdcMax_A_maxval
      link override Signal_Limit/_minval: Value=KOUTP_FrIdcMax_A_minval
      link override Signal_Override/_ovrdflg: Value=KOUTP_FrIdcMax_A_ovrdflg
      link override Signal_Override/_ovrdval: Value=KOUTP_FrIdcMax_A_ovrdval
  VTQD_FrIdcMin_A_Inproc : FVT_lib/outp/OverrideAndLimit  SystemSampleTime=-1  VariantActivationTime=update diagram  Latency=0  AutoFrameSizeCalculation=off
      link override Signal_Limit/_maxval: Value=KOUTP_FrIdcMin_A_maxval
      link override Signal_Limit/_minval: Value=KOUTP_FrIdcMin_A_minval
      link override Signal_Override/_ovrdflg: Value=KOUTP_FrIdcMin_A_ovrdflg
      link override Signal_Override/_ovrdval: Value=KOUTP_FrIdcMin_A_ovrdval
  VTQD_FrRgnDecrSta_flg_Inproc : FVT_lib/outp/OverrideAndLimit  SystemSampleTime=-1  VariantActivationTime=update diagram  Latency=0  AutoFrameSizeCalculation=off
      link override Signal_Limit/_maxval: Value=KOUTP_FrRgnDecrSta_flg_maxval
      link override Signal_Limit/_minval: Value=KOUTP_FrRgnDecrSta_flg_minval
      link override Signal_Override/_ovrdflg: Value=KOUTP_FrRgnDecrSta_flg_ovrdflg
      link override Signal_Override/_ovrdval: Value=KOUTP_FrRgnDecrSta_flg_ovrdval
  VTQD_FrRgnPermSta_flg_Inproc : FVT_lib/outp/OverrideAndLimit  SystemSampleTime=-1  VariantActivationTime=update diagram  Latency=0  AutoFrameSizeCalculation=off
      link override Signal_Limit/_maxval: Value=KOUTP_FrRgnPermSta_flg_maxval
      link override Signal_Limit/_minval: Value=KOUTP_FrRgnPermSta_flg_minval
      link override Signal_Override/_ovrdflg: Value=KOUTP_FrRgnPermSta_flg_ovrdflg
      link override Signal_Override/_ovrdval: Value=KOUTP_FrRgnPermSta_flg_ovrdval
  VTQD_FrUdcMax_V_Inproc : FVT_lib/outp/OverrideAndLimit  SystemSampleTime=-1  VariantActivationTime=update diagram  Latency=0  AutoFrameSizeCalculation=off
      link override Signal_Limit/_maxval: Value=KOUTP_FrUdcMax_V_maxval
      link override Signal_Limit/_minval: Value=KOUTP_FrUdcMax_V_minval
      link override Signal_Override/_ovrdflg: Value=KOUTP_FrUdcMax_V_ovrdflg
      link override Signal_Override/_ovrdval: Value=KOUTP_FrUdcMax_V_ovrdval
  VTQD_FrUdcMin_V_Inproc : FVT_lib/outp/OverrideAndLimit  SystemSampleTime=-1  VariantActivationTime=update diagram  Latency=0  AutoFrameSizeCalculation=off
      link override Signal_Limit/_maxval: Value=KOUTP_FrUdcMin_V_maxval
      link override Signal_Limit/_minval: Value=KOUTP_FrUdcMin_V_minval
      link override Signal_Override/_ovrdflg: Value=KOUTP_FrUdcMin_V_ovrdflg
      link override Signal_Override/_ovrdval: Value=KOUTP_FrUdcMin_V_ovrdval
  VTQD_IVIPwrLockSta_enum_Inproc : FVT_lib/outp/OverrideAndLimit  SystemSampleTime=-1  VariantActivationTime=update diagram  Latency=0  AutoFrameSizeCalculation=off
      link override Signal_Limit/_maxval: Value=KOUTP_IVIPwrLockSta_enum_maxval
      link override Signal_Limit/_minval: Value=KOUTP_IVIPwrLockSta_enum_minval
      link override Signal_Override/_ovrdflg: Value=KOUTP_IVIPwrLockSta_enum_ovrdflg
      link override Signal_Override/_ovrdval: Value=KOUTP_IVIPwrLockSta_enum_ovrdval
  VTQD_OPDHoldLamp_flg_Inproc : FVT_lib/outp/OverrideAndLimit  SystemSampleTime=-1  VariantActivationTime=update diagram  Latency=0  AutoFrameSizeCalculation=off
      link override Signal_Limit/_maxval: Value=KOUTP_OPDHoldLamp_flg_maxval
      link override Signal_Limit/_minval: Value=KOUTP_OPDHoldLamp_flg_minval
      link override Signal_Override/_ovrdflg: Value=KOUTP_OPDHoldLamp_flg_ovrdflg
      link override Signal_Override/_ovrdval: Value=KOUTP_OPDHoldLamp_flg_ovrdval
  VTQD_PButtonSta_enum_Inproc : FVT_lib/outp/OverrideAndLimit  SystemSampleTime=-1  VariantActivationTime=update diagram  Latency=0  AutoFrameSizeCalculation=off
      link override Signal_Limit/_maxval: Value=KOUTP_PButtonSta_enum_maxval
      link override Signal_Limit/_minval: Value=KOUTP_PButtonSta_enum_minval
      link override Signal_Override/_ovrdflg: Value=KOUTP_PButtonSta_enum_ovrdflg
      link override Signal_Override/_ovrdval: Value=KOUTP_PButtonSta_enum_ovrdval
  VTQD_PTCSPermSta_flg_Inproc : FVT_lib/outp/OverrideAndLimit  SystemSampleTime=-1  VariantActivationTime=update diagram  Latency=0  AutoFrameSizeCalculation=off
      link override Signal_Limit/_maxval: Value=KOUTP_PTCSPermSta_flg_maxval
      link override Signal_Limit/_minval: Value=KOUTP_PTCSPermSta_flg_minval
      link override Signal_Override/_ovrdflg: Value=KOUTP_PTCSPermSta_flg_ovrdflg
      link override Signal_Override/_ovrdval: Value=KOUTP_PTCSPermSta_flg_ovrdval
  VTQD_ParkRequest_flg_Inproc : FVT_lib/outp/OverrideAndLimit  SystemSampleTime=-1  VariantActivationTime=update diagram  Latency=0  AutoFrameSizeCalculation=off
      link override Signal_Limit/_maxval: Value=KOUTP_ParkRequest_flg_maxval
      link override Signal_Limit/_minval: Value=KOUTP_ParkRequest_flg_minval
      link override Signal_Override/_ovrdflg: Value=KOUTP_ParkRequest_flg_ovrdflg
      link override Signal_Override/_ovrdval: Value=KOUTP_ParkRequest_flg_ovrdval
  VTQD_ReBrakeLPReq_flg_Inproc : FVT_lib/outp/OverrideAndLimit  SystemSampleTime=-1  VariantActivationTime=update diagram  Latency=0  AutoFrameSizeCalculation=off
      link override Signal_Limit/_maxval: Value=KOUTP_ReBrakeLPReq_flg_maxval
      link override Signal_Limit/_minval: Value=KOUTP_ReBrakeLPReq_flg_minval
      link override Signal_Override/_ovrdflg: Value=KOUTP_ReBrakeLPReq_flg_ovrdflg
      link override Signal_Override/_ovrdval: Value=KOUTP_ReBrakeLPReq_flg_ovrdval
  VTQD_RgnAbnorSta_flg_Inproc : FVT_lib/outp/OverrideAndLimit  SystemSampleTime=-1  VariantActivationTime=update diagram  Latency=0  AutoFrameSizeCalculation=off
      link override Signal_Limit/_maxval: Value=KOUTP_RgnAbnorSta_flg_maxval
      link override Signal_Limit/_minval: Value=KOUTP_RgnAbnorSta_flg_minval
      link override Signal_Override/_ovrdflg: Value=KOUTP_RgnAbnorSta_flg_ovrdflg
      link override Signal_Override/_ovrdval: Value=KOUTP_RgnAbnorSta_flg_ovrdval
  VTQD_RrActvDmpDisabReq_flg_Inproc : FVT_lib/outp/OverrideAndLimit  SystemSampleTime=-1  VariantActivationTime=update diagram  Latency=0  AutoFrameSizeCalculation=off
      link override Signal_Limit/_maxval: Value=KOUTP_RrActvDmpDisabReq_flg_maxval
      link override Signal_Limit/_minval: Value=KOUTP_RrActvDmpDisabReq_flg_minval
      link override Signal_Override/_ovrdflg: Value=KOUTP_RrActvDmpDisabReq_flg_ovrdflg
      link override Signal_Override/_ovrdval: Value=KOUTP_RrActvDmpDisabReq_flg_ovrdval
  VTQD_RrEDUActTq_Nm_Inproc : FVT_lib/outp/OverrideAndLimit  SystemSampleTime=-1  VariantActivationTime=update diagram  Latency=0  AutoFrameSizeCalculation=off
      link override Signal_Limit/_maxval: Value=KOUTP_RrEDUActTq_Nm_maxval
      link override Signal_Limit/_minval: Value=KOUTP_RrEDUActTq_Nm_minval
      link override Signal_Override/_ovrdflg: Value=KOUTP_RrEDUActTq_Nm_ovrdflg
      link override Signal_Override/_ovrdval: Value=KOUTP_RrEDUActTq_Nm_ovrdval
  VTQD_RrEDUAvailBrkRgnTqV_flg_Inproc : FVT_lib/outp/OverrideAndLimit  SystemSampleTime=-1  VariantActivationTime=update diagram  Latency=0  AutoFrameSizeCalculation=off
      link override Signal_Limit/_maxval: Value=KOUTP_RrEDUAvailBrkRgnTqV_flg_maxval
      link override Signal_Limit/_minval: Value=KOUTP_RrEDUAvailBrkRgnTqV_flg_minval
      link override Signal_Override/_ovrdflg: Value=KOUTP_RrEDUAvailBrkRgnTqV_flg_ovrdflg
      link override Signal_Override/_ovrdval: Value=KOUTP_RrEDUAvailBrkRgnTqV_flg_ovrdval
  VTQD_RrEDUAvailBrkRgnTq_Nm_Inproc : FVT_lib/outp/OverrideAndLimit  SystemSampleTime=-1  VariantActivationTime=update diagram  Latency=0  AutoFrameSizeCalculation=off
      link override Signal_Limit/_maxval: Value=KOUTP_RrEDUAvailBrkRgnTq_Nm_maxval
      link override Signal_Limit/_minval: Value=KOUTP_RrEDUAvailBrkRgnTq_Nm_minval
      link override Signal_Override/_ovrdflg: Value=KOUTP_RrEDUAvailBrkRgnTq_Nm_ovrdflg
      link override Signal_Override/_ovrdval: Value=KOUTP_RrEDUAvailBrkRgnTq_Nm_ovrdval
  VTQD_RrEDURolRgnTq_Nm_Inproc : FVT_lib/outp/OverrideAndLimit  SystemSampleTime=-1  VariantActivationTime=update diagram  Latency=0  AutoFrameSizeCalculation=off
      link override Signal_Limit/_maxval: Value=KOUTP_RrEDURolRgnTq_Nm_maxval
      link override Signal_Limit/_minval: Value=KOUTP_RrEDURolRgnTq_Nm_minval
      link override Signal_Override/_ovrdflg: Value=KOUTP_RrEDURolRgnTq_Nm_ovrdflg
      link override Signal_Override/_ovrdval: Value=KOUTP_RrEDURolRgnTq_Nm_ovrdval
  VTQD_RrEDUSpdValid_flg_Inproc : FVT_lib/outp/OverrideAndLimit  SystemSampleTime=-1  VariantActivationTime=update diagram  Latency=0  AutoFrameSizeCalculation=off
      link override Signal_Limit/_maxval: Value=KOUTP_RrEDUSpdValid_flg_maxval
      link override Signal_Limit/_minval: Value=KOUTP_RrEDUSpdValid_flg_minval
      link override Signal_Override/_ovrdflg: Value=KOUTP_RrEDUSpdValid_flg_ovrdflg
      link override Signal_Override/_ovrdval: Value=KOUTP_RrEDUSpdValid_flg_ovrdval
  VTQD_RrEDUSpd_rpm_Inproc : FVT_lib/outp/OverrideAndLimit  SystemSampleTime=-1  VariantActivationTime=update diagram  Latency=0  AutoFrameSizeCalculation=off
      link override Signal_Limit/_maxval: Value=KOUTP_RrEDUSpd_rpm_maxval
      link override Signal_Limit/_minval: Value=KOUTP_RrEDUSpd_rpm_minval
      link override Signal_Override/_ovrdflg: Value=KOUTP_RrEDUSpd_rpm_ovrdflg
      link override Signal_Override/_ovrdval: Value=KOUTP_RrEDUSpd_rpm_ovrdval
  VTQD_RrIdcMax_A_Inproc : FVT_lib/outp/OverrideAndLimit  SystemSampleTime=-1  VariantActivationTime=update diagram  Latency=0  AutoFrameSizeCalculation=off
      link override Signal_Limit/_maxval: Value=KOUTP_RrIdcMax_A_maxval
      link override Signal_Limit/_minval: Value=KOUTP_RrIdcMax_A_minval
      link override Signal_Override/_ovrdflg: Value=KOUTP_RrIdcMax_A_ovrdflg
      link override Signal_Override/_ovrdval: Value=KOUTP_RrIdcMax_A_ovrdval
  VTQD_RrIdcMin_A_Inproc : FVT_lib/outp/OverrideAndLimit  SystemSampleTime=-1  VariantActivationTime=update diagram  Latency=0  AutoFrameSizeCalculation=off
      link override Signal_Limit/_maxval: Value=KOUTP_RrIdcMin_A_maxval
      link override Signal_Limit/_minval: Value=KOUTP_RrIdcMin_A_minval
      link override Signal_Override/_ovrdflg: Value=KOUTP_RrIdcMin_A_ovrdflg
      link override Signal_Override/_ovrdval: Value=KOUTP_RrIdcMin_A_ovrdval
  VTQD_RrRgnDecrSta_flg_Inproc : FVT_lib/outp/OverrideAndLimit  SystemSampleTime=-1  VariantActivationTime=update diagram  Latency=0  AutoFrameSizeCalculation=off
      link override Signal_Limit/_maxval: Value=KOUTP_RrRgnDecrSta_flg_maxval
      link override Signal_Limit/_minval: Value=KOUTP_RrRgnDecrSta_flg_minval
      link override Signal_Override/_ovrdflg: Value=KOUTP_RrRgnDecrSta_flg_ovrdflg
      link override Signal_Override/_ovrdval: Value=KOUTP_RrRgnDecrSta_flg_ovrdval
  VTQD_RrRgnPermSta_flg_Inproc : FVT_lib/outp/OverrideAndLimit  SystemSampleTime=-1  VariantActivationTime=update diagram  Latency=0  AutoFrameSizeCalculation=off
      link override Signal_Limit/_maxval: Value=KOUTP_RrRgnPermSta_flg_maxval
      link override Signal_Limit/_minval: Value=KOUTP_RrRgnPermSta_flg_minval
      link override Signal_Override/_ovrdflg: Value=KOUTP_RrRgnPermSta_flg_ovrdflg
      link override Signal_Override/_ovrdval: Value=KOUTP_RrRgnPermSta_flg_ovrdval
  VTQD_RrUdcMax_V_Inproc : FVT_lib/outp/OverrideAndLimit  SystemSampleTime=-1  VariantActivationTime=update diagram  Latency=0  AutoFrameSizeCalculation=off
      link override Signal_Limit/_maxval: Value=KOUTP_RrUdcMax_V_maxval
      link override Signal_Limit/_minval: Value=KOUTP_RrUdcMax_V_minval
      link override Signal_Override/_ovrdflg: Value=KOUTP_RrUdcMax_V_ovrdflg
      link override Signal_Override/_ovrdval: Value=KOUTP_RrUdcMax_V_ovrdval
  VTQD_RrUdcMin_V_Inproc : FVT_lib/outp/OverrideAndLimit  SystemSampleTime=-1  VariantActivationTime=update diagram  Latency=0  AutoFrameSizeCalculation=off
      link override Signal_Limit/_maxval: Value=KOUTP_RrUdcMin_V_maxval
      link override Signal_Limit/_minval: Value=KOUTP_RrUdcMin_V_minval
      link override Signal_Override/_ovrdflg: Value=KOUTP_RrUdcMin_V_ovrdflg
      link override Signal_Override/_ovrdval: Value=KOUTP_RrUdcMin_V_ovrdval
  VTQD_ShiftGearPosn_enum_Inproc : FVT_lib/outp/OverrideAndLimit  SystemSampleTime=-1  VariantActivationTime=update diagram  Latency=0  AutoFrameSizeCalculation=off
      link override Signal_Limit/_maxval: Value=KOUTP_ShiftGearPosn_enum_maxval
      link override Signal_Limit/_minval: Value=KOUTP_ShiftGearPosn_enum_minval
      link override Signal_Override/_ovrdflg: Value=KOUTP_ShiftGearPosn_enum_ovrdflg
      link override Signal_Override/_ovrdval: Value=KOUTP_ShiftGearPosn_enum_ovrdval
  VTQD_TqSourceFr_enum_Inproc : FVT_lib/outp/OverrideAndLimit  SystemSampleTime=-1  VariantActivationTime=update diagram  Latency=0  AutoFrameSizeCalculation=off
      link override Signal_Limit/_maxval: Value=KOUTP_TqSourceFr_enum_maxval
      link override Signal_Limit/_minval: Value=KOUTP_TqSourceFr_enum_minval
      link override Signal_Override/_ovrdflg: Value=KOUTP_TqSourceFr_enum_ovrdflg
      link override Signal_Override/_ovrdval: Value=KOUTP_TqSourceFr_enum_ovrdval
  VTQD_TqSourceRr_enum_Inproc : FVT_lib/outp/OverrideAndLimit  SystemSampleTime=-1  VariantActivationTime=update diagram  Latency=0  AutoFrameSizeCalculation=off
      link override Signal_Limit/_maxval: Value=KOUTP_TqSourceRr_enum_maxval
      link override Signal_Limit/_minval: Value=KOUTP_TqSourceRr_enum_minval
      link override Signal_Override/_ovrdflg: Value=KOUTP_TqSourceRr_enum_ovrdflg
      link override Signal_Override/_ovrdval: Value=KOUTP_TqSourceRr_enum_ovrdval
  VTQD_VehActSpd_kph_Inproc : FVT_lib/outp/OverrideAndLimit  SystemSampleTime=-1  VariantActivationTime=update diagram  Latency=0  AutoFrameSizeCalculation=off
      link override Signal_Limit/_maxval: Value=KOUTP_VehActSpd_kph_maxval
      link override Signal_Limit/_minval: Value=KOUTP_VehActSpd_kph_minval
      link override Signal_Override/_ovrdflg: Value=KOUTP_VehActSpd_kph_ovrdflg
      link override Signal_Override/_ovrdval: Value=KOUTP_VehActSpd_kph_ovrdval
  VTQR_FrTMTqReq_Nm_Inproc : FVT_lib/outp/OverrideAndLimit  SystemSampleTime=-1  VariantActivationTime=update diagram  Latency=0  AutoFrameSizeCalculation=off
      link override Signal_Limit/_maxval: Value=KOUTP_FrTMTqReq_Nm_maxval
      link override Signal_Limit/_minval: Value=KOUTP_FrTMTqReq_Nm_minval
      link override Signal_Override/_ovrdflg: Value=KOUTP_FrTMTqReq_Nm_ovrdflg
      link override Signal_Override/_ovrdval: Value=KOUTP_FrTMTqReq_Nm_ovrdval
  VTQR_RrTMTqReq_Nm_Inproc : FVT_lib/outp/OverrideAndLimit  SystemSampleTime=-1  VariantActivationTime=update diagram  Latency=0  AutoFrameSizeCalculation=off
      link override Signal_Limit/_maxval: Value=KOUTP_RrTMTqReq_Nm_maxval
      link override Signal_Limit/_minval: Value=KOUTP_RrTMTqReq_Nm_minval
      link override Signal_Override/_ovrdflg: Value=KOUTP_RrTMTqReq_Nm_ovrdflg
      link override Signal_Override/_ovrdval: Value=KOUTP_RrTMTqReq_Nm_ovrdval
  VV2L_ReqOBCV2LEna_enum_Inproc : FVT_lib/outp/OverrideAndLimit  SystemSampleTime=-1  VariantActivationTime=update diagram  Latency=0  AutoFrameSizeCalculation=off
      link override Signal_Limit/_maxval: Value=KOUTP_ReqOBCV2LEna_enum_maxval
      link override Signal_Limit/_minval: Value=KOUTP_ReqOBCV2LEna_enum_minval
      link override Signal_Override/_ovrdflg: Value=KOUTP_ReqOBCV2LEna_enum_ovrdflg
      link override Signal_Override/_ovrdval: Value=KOUTP_ReqOBCV2LEna_enum_ovrdval
  VV2L_ReqV2LIVIPopup_enum_Inproc : FVT_lib/outp/OverrideAndLimit  SystemSampleTime=-1  VariantActivationTime=update diagram  Latency=0  AutoFrameSizeCalculation=off
      link override Signal_Limit/_maxval: Value=KOUTP_ReqV2LIVIPopup_enum_maxval
      link override Signal_Limit/_minval: Value=KOUTP_ReqV2LIVIPopup_enum_minval
      link override Signal_Override/_ovrdflg: Value=KOUTP_ReqV2LIVIPopup_enum_ovrdflg
      link override Signal_Override/_ovrdval: Value=KOUTP_ReqV2LIVIPopup_enum_ovrdval
  VVMC_ACCCtrlAvail_flg_Inproc : FVT_lib/outp/OverrideAndLimit  SystemSampleTime=-1  VariantActivationTime=update diagram  Latency=0  AutoFrameSizeCalculation=off
      link override Signal_Limit/_maxval: Value=KOUTP_ACCCtrlAvail_flg_maxval
      link override Signal_Limit/_minval: Value=KOUTP_ACCCtrlAvail_flg_minval
      link override Signal_Override/_ovrdflg: Value=KOUTP_ACCCtrlAvail_flg_ovrdflg
      link override Signal_Override/_ovrdval: Value=KOUTP_ACCCtrlAvail_flg_ovrdval
  VVMC_ACCPedalOvrd_flg_Inproc : FVT_lib/outp/OverrideAndLimit  SystemSampleTime=-1  VariantActivationTime=update diagram  Latency=0  AutoFrameSizeCalculation=off
      link override Signal_Limit/_maxval: Value=KOUTP_ACCPedalOvrd_flg_maxval
      link override Signal_Limit/_minval: Value=KOUTP_ACCPedalOvrd_flg_minval
      link override Signal_Override/_ovrdflg: Value=KOUTP_ACCPedalOvrd_flg_ovrdflg
      link override Signal_Override/_ovrdval: Value=KOUTP_ACCPedalOvrd_flg_ovrdval
  VVMC_APSActive_flg_Inproc : FVT_lib/outp/OverrideAndLimit  SystemSampleTime=-1  VariantActivationTime=update diagram  Latency=0  AutoFrameSizeCalculation=off
      link override Signal_Limit/_maxval: Value=KOUTP_APSActive_flg_maxval
      link override Signal_Limit/_minval: Value=KOUTP_APSActive_flg_minval
      link override Signal_Override/_ovrdflg: Value=KOUTP_APSActive_flg_ovrdflg
      link override Signal_Override/_ovrdval: Value=KOUTP_APSActive_flg_ovrdval
  VVMC_APSCtrlAvail_flg_Inproc : FVT_lib/outp/OverrideAndLimit  SystemSampleTime=-1  VariantActivationTime=update diagram  Latency=0  AutoFrameSizeCalculation=off
      link override Signal_Limit/_maxval: Value=KOUTP_APSCtrlAvail_flg_maxval
      link override Signal_Limit/_minval: Value=KOUTP_APSCtrlAvail_flg_minval
      link override Signal_Override/_ovrdflg: Value=KOUTP_APSCtrlAvail_flg_ovrdflg
      link override Signal_Override/_ovrdval: Value=KOUTP_APSCtrlAvail_flg_ovrdval
  VVMC_APSDecReqA_flg_Inproc : FVT_lib/outp/OverrideAndLimit  SystemSampleTime=-1  VariantActivationTime=update diagram  Latency=0  AutoFrameSizeCalculation=off
      link override Signal_Limit/_maxval: Value=KOUTP_APSDecReqA_flg_maxval
      link override Signal_Limit/_minval: Value=KOUTP_APSDecReqA_flg_minval
      link override Signal_Override/_ovrdflg: Value=KOUTP_APSDecReqA_flg_ovrdflg
      link override Signal_Override/_ovrdval: Value=KOUTP_APSDecReqA_flg_ovrdval
  VVMC_APSDecReq_mps2_Inproc : FVT_lib/outp/OverrideAndLimit  SystemSampleTime=-1  VariantActivationTime=update diagram  Latency=0  AutoFrameSizeCalculation=off
      link override Signal_Limit/_maxval: Value=KOUTP_APSDecReq_mps2_maxval
      link override Signal_Limit/_minval: Value=KOUTP_APSDecReq_mps2_minval
      link override Signal_Override/_ovrdflg: Value=KOUTP_APSDecReq_mps2_ovrdflg
      link override Signal_Override/_ovrdval: Value=KOUTP_APSDecReq_mps2_ovrdval
  VVMC_APSReq_enum_Inproc : FVT_lib/outp/OverrideAndLimit  SystemSampleTime=-1  VariantActivationTime=update diagram  Latency=0  AutoFrameSizeCalculation=off
      link override Signal_Limit/_maxval: Value=KOUTP_APSReq_enum_maxval
      link override Signal_Limit/_minval: Value=KOUTP_APSReq_enum_minval
      link override Signal_Override/_ovrdflg: Value=KOUTP_APSReq_enum_ovrdflg
      link override Signal_Override/_ovrdval: Value=KOUTP_APSReq_enum_ovrdval
  VVMC_APSStaSys_enum_Inproc : FVT_lib/outp/OverrideAndLimit  SystemSampleTime=-1  VariantActivationTime=update diagram  Latency=0  AutoFrameSizeCalculation=off
      link override Signal_Limit/_maxval: Value=KOUTP_APSStaSys_enum_maxval
      link override Signal_Limit/_minval: Value=KOUTP_APSStaSys_enum_minval
      link override Signal_Override/_ovrdflg: Value=KOUTP_APSStaSys_enum_ovrdflg
      link override Signal_Override/_ovrdval: Value=KOUTP_APSStaSys_enum_ovrdval
  VVMC_CAASActive_flg_Inproc : FVT_lib/outp/OverrideAndLimit  SystemSampleTime=-1  VariantActivationTime=update diagram  Latency=0  AutoFrameSizeCalculation=off
      link override Signal_Limit/_maxval: Value=KOUTP_CAASActive_flg_maxval
      link override Signal_Limit/_minval: Value=KOUTP_CAASActive_flg_minval
      link override Signal_Override/_ovrdflg: Value=KOUTP_CAASActive_flg_ovrdflg
      link override Signal_Override/_ovrdval: Value=KOUTP_CAASActive_flg_ovrdval
  VVMC_CAASCtrlAvail_flg_Inproc : FVT_lib/outp/OverrideAndLimit  SystemSampleTime=-1  VariantActivationTime=update diagram  Latency=0  AutoFrameSizeCalculation=off
      link override Signal_Limit/_maxval: Value=KOUTP_CAASCtrlAvail_flg_maxval
      link override Signal_Limit/_minval: Value=KOUTP_CAASCtrlAvail_flg_minval
      link override Signal_Override/_ovrdflg: Value=KOUTP_CAASCtrlAvail_flg_ovrdflg
      link override Signal_Override/_ovrdval: Value=KOUTP_CAASCtrlAvail_flg_ovrdval
  VVMC_CCCtrlSta_enum_Inproc : FVT_lib/outp/OverrideAndLimit  SystemSampleTime=-1  VariantActivationTime=update diagram  Latency=0  AutoFrameSizeCalculation=off
      link override Signal_Limit/_maxval: Value=KOUTP_CCCtrlSta_enum_maxval
      link override Signal_Limit/_minval: Value=KOUTP_CCCtrlSta_enum_minval
      link override Signal_Override/_ovrdflg: Value=KOUTP_CCCtrlSta_enum_ovrdflg
      link override Signal_Override/_ovrdval: Value=KOUTP_CCCtrlSta_enum_ovrdval
  VVMC_CCMSASpdWar_flg_Inproc : FVT_lib/outp/OverrideAndLimit  SystemSampleTime=-1  VariantActivationTime=update diagram  Latency=0  AutoFrameSizeCalculation=off
      link override Signal_Limit/_maxval: Value=KOUTP_CCMSASpdWar_flg_maxval
      link override Signal_Limit/_minval: Value=KOUTP_CCMSASpdWar_flg_minval
      link override Signal_Override/_ovrdflg: Value=KOUTP_CCMSASpdWar_flg_ovrdflg
      link override Signal_Override/_ovrdval: Value=KOUTP_CCMSASpdWar_flg_ovrdval
  VVMC_ExtraMSACtrlSta_enum_Inproc : FVT_lib/outp/OverrideAndLimit  SystemSampleTime=-1  VariantActivationTime=update diagram  Latency=0  AutoFrameSizeCalculation=off
      link override Signal_Limit/_maxval: Value=KOUTP_ExtraMSACtrlSta_enum_maxval
      link override Signal_Limit/_minval: Value=KOUTP_ExtraMSACtrlSta_enum_minval
      link override Signal_Override/_ovrdflg: Value=KOUTP_ExtraMSACtrlSta_enum_ovrdflg
      link override Signal_Override/_ovrdval: Value=KOUTP_ExtraMSACtrlSta_enum_ovrdval
  VVMC_IMUEnaCmd_flg_Inproc : FVT_lib/outp/OverrideAndLimit  SystemSampleTime=-1  VariantActivationTime=update diagram  Latency=0  AutoFrameSizeCalculation=off
      link override Signal_Limit/_maxval: Value=KOUTP_IMUEnaCmd_flg_maxval
      link override Signal_Limit/_minval: Value=KOUTP_IMUEnaCmd_flg_minval
      link override Signal_Override/_ovrdflg: Value=KOUTP_IMUEnaCmd_flg_ovrdflg
      link override Signal_Override/_ovrdval: Value=KOUTP_IMUEnaCmd_flg_ovrdval
  VVMC_MSACtrlSta_enum_Inproc : FVT_lib/outp/OverrideAndLimit  SystemSampleTime=-1  VariantActivationTime=update diagram  Latency=0  AutoFrameSizeCalculation=off
      link override Signal_Limit/_maxval: Value=KOUTP_MSACtrlSta_enum_maxval
      link override Signal_Limit/_minval: Value=KOUTP_MSACtrlSta_enum_minval
      link override Signal_Override/_ovrdflg: Value=KOUTP_MSACtrlSta_enum_ovrdflg
      link override Signal_Override/_ovrdval: Value=KOUTP_MSACtrlSta_enum_ovrdval
  VOUTP_HVTHCMSysAvail_enum : Outport
  VOUTP_LVBattVoltSta_enum : Outport  Port=2
  VOUTP_VehHVPwrAvail4THCM_W : Outport  Port=3
  VOUTP_VehSpeed_kph : Outport  Port=4
  VOUTP_VehSpeedTimeOut_flg : Outport  Port=5
  VOUTP_FSOffSw_enum : Outport  Port=6
  VOUTP_FSOffSwTimeOut_flg : Outport  Port=7
  VOUTP_ChrgPlugSta_enum : Outport  Port=8
  VOUTP_PASDRMR_cm : Outport  Port=9
  VOUTP_PASDRML_cm : Outport  Port=10
  VOUTP_PASDRCR_cm : Outport  Port=11
  VOUTP_PASDRCL_cm : Outport  Port=12
  VOUTP_PASDFMR_cm : Outport  Port=13
  VOUTP_PASDFML_cm : Outport  Port=14
  VOUTP_PASDFCR_cm : Outport  Port=15
  VOUTP_PASDFCL_cm : Outport  Port=16
  VOUTP_APSDRLR_cm : Outport  Port=17
  VOUTP_APSDRLL_cm : Outport  Port=18
  VOUTP_APSDFLR_cm : Outport  Port=19
  VOUTP_APSDFLL_cm : Outport  Port=20
  VOUTP_PASAFCL_enum : Outport  Port=21
  VOUTP_PASARMR_enum : Outport  Port=22
  VOUTP_PASARML_enum : Outport  Port=23
  VOUTP_PASARCR_enum : Outport  Port=24
  VOUTP_PASARCL_enum : Outport  Port=25
  VOUTP_PASAFMR_enum : Outport  Port=26
  VOUTP_PASAFML_enum : Outport  Port=27
  VOUTP_PASAFCR_enum : Outport  Port=28
  VOUTP_USSStaRMR_flg : Outport  Port=29
  VOUTP_USSStaRML_flg : Outport  Port=30
  VOUTP_USSStaRLR_flg : Outport  Port=31
  VOUTP_USSStaRLL_flg : Outport  Port=32
  VOUTP_USSStaRCR_flg : Outport  Port=33
  VOUTP_USSStaRCL_flg : Outport  Port=34
  VOUTP_USSStaFMR_flg : Outport  Port=35
  VOUTP_USSStaFML_flg : Outport  Port=36
  VOUTP_USSStaFLR_flg : Outport  Port=37
  VOUTP_USSStaFLL_flg : Outport  Port=38
  VOUTP_USSStaFCR_flg : Outport  Port=39
  VOUTP_USSStaFCL_flg : Outport  Port=40
  VOUTP_Chime_enum : Outport  Port=41
  VOUTP_SNSRLayout_enum : Outport  Port=42
  VOUTP_StaFSya_flg : Outport  Port=43
  VOUTP_ModOperation_enum : Outport  Port=44
  VOUTP_BrkPedalPos_pct : Outport  Port=45
  VOUTP_BrkPedalPosTimeOut_flg : Outport  Port=46
  VOUTP_LFRawWhlSpeed_kph : Outport  Port=47
  VOUTP_LFRawWhlSpeedTimeOut_flg : Outport  Port=48
  VOUTP_RFRawWhlSpeed_kph : Outport  Port=49
  VOUTP_RFRawWhlSpeedTimeOut_flg : Outport  Port=50
  VOUTP_LRRawWhlSpeed_kph : Outport  Port=51
  VOUTP_LRRawWhlSpeedTimeOut_flg : Outport  Port=52
  VOUTP_RRRawWhlSpeed_kph : Outport  Port=53
  VOUTP_RRRawWhlSpeedTimeOut_flg : Outport  Port=54
  VOUTP_LFRawWhlSpeedV_flg : Outport  Port=55
  VOUTP_LFRawWhlSpeedVTimeOut_flg : Outport  Port=56
  VOUTP_RFRawWhlSpeedV_flg : Outport  Port=57
  VOUTP_RFRawWhlSpeedVTimeOut_flg : Outport  Port=58
  VOUTP_LRRawWhlSpeedV_flg : Outport  Port=59
  VOUTP_LRRawWhlSpeedVTimeOut_flg : Outport  Port=60
  VOUTP_RRRawWhlSpeedV_flg : Outport  Port=61
  VOUTP_RRRawWhlSpeedVTimeOut_flg : Outport  Port=62
  VOUTP_LFWhlRotDir_enum : Outport  Port=63
  VOUTP_LFWhlRotDirTimeOut_flg : Outport  Port=64
  VOUTP_RFWhlRotDir_enum : Outport  Port=65
  VOUTP_RFWhlRotDirTimeOut_flg : Outport  Port=66
  VOUTP_LRWhlRotDir_enum : Outport  Port=67
  VOUTP_LRWhlRotDirTimeOut_flg : Outport  Port=68
  VOUTP_RRWhlRotDir_enum : Outport  Port=69
  VOUTP_RRWhlRotDirTimeOut_flg : Outport  Port=70
  VOUTP_LFPulseCountV_flg : Outport  Port=71
  VOUTP_LFPulseCountVTimeOut_flg : Outport  Port=72
  VOUTP_RFPulseCountV_flg : Outport  Port=73
  VOUTP_RFPulseCountVTimeOut_flg : Outport  Port=74
  VOUTP_LRPulseCountV_flg : Outport  Port=75
  VOUTP_LRPulseCountVTimeOut_flg : Outport  Port=76
  VOUTP_RRPulseCountV_flg : Outport  Port=77
  VOUTP_RRPulseCountVTimeOut_flg : Outport  Port=78
  VOUTP_LFPulseCount_enum : Outport  Port=79
  VOUTP_LFPulseCountTimeOut_flg : Outport  Port=80
  VOUTP_RFPulseCount_enum : Outport  Port=81
  VOUTP_RFPulseCountTimeOut_flg : Outport  Port=82
  VOUTP_LRPulseCount_enum : Outport  Port=83
  VOUTP_LRPulseCountTimeOut_flg : Outport  Port=84
  VOUTP_RRPulseCount_enum : Outport  Port=85
  VOUTP_RRPulseCountTimeOut_flg : Outport  Port=86
  VOUTP_ShifterHandleCmd_enum : Outport  Port=87
  VOUTP_ShifterHandleCmdTimeOut_flg : Outport  Port=88
  VOUTP_DriIntend_enum : Outport  Port=89
  VOUTP_DriIntendTimeOut_flg : Outport  Port=90
  VOUTP_EPSAOIControl_enum : Outport  Port=91
  VOUTP_EPSAOIControlTimeOut_flg : Outport  Port=92
  VOUTP_SASAngle_Deg : Outport  Port=93
  VOUTP_SASAngleTimeOut_flg : Outport  Port=94
  VOUTP_SASSpeed_degps : Outport  Port=95
  VOUTP_SASSpeedTimeOut_flg : Outport  Port=96
  VOUTP_SASSpeedValid_flg : Outport  Port=97
  VOUTP_SASSpeedValidTimeOut_flg : Outport  Port=98
  VOUTP_SASCAL_flg : Outport  Port=99
  VOUTP_SASCALTimeOut_flg : Outport  Port=100
  VOUTP_SASV_flg : Outport  Port=101
  VOUTP_SASVTimeOut_flg : Outport  Port=102
  VOUTP_GRADE_Deg : Outport  Port=103
  VOUTP_GRADETimeOut_flg : Outport  Port=104
  VOUTP_YawRate_degps : Outport  Port=105
  VOUTP_YawRateTimeOut_flg : Outport  Port=106
  VOUTP_LatAccel_Gps : Outport  Port=107
  VOUTP_LatAccelTimeOut_flg : Outport  Port=108
  VOUTP_LongAccel_Gps : Outport  Port=109
  VOUTP_LongAccelTimeOut_flg : Outport  Port=110
  VOUTP_MCPressure_bar : Outport  Port=111
  VOUTP_MCPressureTimeOut_flg : Outport  Port=112
  VOUTP_YawRateV_flg : Outport  Port=113
  VOUTP_YawRateVTimeOut_flg : Outport  Port=114
  VOUTP_LatAccelV_flg : Outport  Port=115
  VOUTP_LatAccelVTimeOut_flg : Outport  Port=116
  VOUTP_LongAccelV_flg : Outport  Port=117
  VOUTP_LongAccelVTimeOut_flg : Outport  Port=118
  VOUTP_MCPressureV_bar : Outport  Port=119
  VOUTP_MCPressureVTimeOut_flg : Outport  Port=120
  VOUTP_BrkSwSta_flg : Outport  Port=121
  VOUTP_BrkSwStaTimeOut_flg : Outport  Port=122
  VOUTP_BrkSwV_flg : Outport  Port=123
  VOUTP_BrkSwVTimeOut_flg : Outport  Port=124
  VOUTP_ESCStandstill_flg : Outport  Port=125
  VOUTP_ESCStandstillTimeOut_flg : Outport  Port=126
  VOUTP_ESCAPSSta_enum : Outport  Port=127
  VOUTP_ESCAPSStaTimeOut_flg : Outport  Port=128
  VOUTP_EPBExtReleaseAvail_flg : Outport  Port=129
  VOUTP_EPBExtReleaseAvailTimeOut_flg : Outport  Port=130
  VOUTP_EPBExtApplyAvail_flg : Outport  Port=131
  VOUTP_EPBExtApplyAvailTimeOut_flg : Outport  Port=132
  VOUTP_EPBErrSta_enum : Outport  Port=133
  VOUTP_EPBErrStaTimeOut_flg : Outport  Port=134
  VOUTP_EPBSta_enum : Outport  Port=135
  VOUTP_EPBStaTimeOut_flg : Outport  Port=136
  VOUTP_AVMparkingcancel_enum : Outport  Port=137
  VOUTP_AVMparkingcancelTimeOut_flg : Outport  Port=138
  VOUTP_AVMparkingexcute_enum : Outport  Port=139
  VOUTP_AVMparkingexcuteTimeOut_flg : Outport  Port=140
  VOUTP_AVMParkingmode_enum : Outport  Port=141
  VOUTP_AVMParkingmodeTimeOut_flg : Outport  Port=142
  VOUTP_AVMErrSTA_flg : Outport  Port=143
  VOUTP_AVMErrSTATimeOut_flg : Outport  Port=144
  VOUTP_IVIStatus_flg : Outport  Port=145
  VOUTP_IVIStatusTimeOut_flg : Outport  Port=146
  VOUTP_CAASSw_enum : Outport  Port=147
  VOUTP_CAASSwTimeOut_flg : Outport  Port=148
  VOUTP_IVIScreen_enum : Outport  Port=149
  VOUTP_IVIScreenTimeOut_flg : Outport  Port=150
  VOUTP_ABSActive_flg : Outport  Port=151
  VOUTP_ABSActiveTimeOut_flg : Outport  Port=152
  VOUTP_TCSActive_flg : Outport  Port=153
  VOUTP_TCSActiveTimeOut_flg : Outport  Port=154
  VOUTP_DriverSeatBeltCmd_flg : Outport  Port=155
  VOUTP_DriverSeatBeltCmdTimeOut_flg : Outport  Port=156
  VOUTP_APSProgressPCT_pct : Outport  Port=157
  VOUTP_APSRQDisplay_enum : Outport  Port=158
  VOUTP_APSSWVer_enum : Outport  Port=159
  VOUTP_APSHWVer_enum : Outport  Port=160
  VOUTP_APSExitCondition_enum : Outport  Port=161
  VOUTP_APSAngleTarget_Deg : Outport  Port=162
  VOUTP_APSVRqEPASCtrl_flg : Outport  Port=163
  VOUTP_APSRqEPASCtrl_flg : Outport  Port=164
  VOUTP_CAASSta_enum : Outport  Port=165
  VOUTP_AntitheftSta_enum : Outport  Port=166
  VOUTP_TailgateRemote_enum : Outport  Port=167
  VOUTP_HornCtrl_flg : Outport  Port=168
  VOUTP_AllDoorSW_flg : Outport  Port=169
  VOUTP_BCMDoorLockSta_flg : Outport  Port=170
  VOUTP_AntitheftSeatFlod_flg : Outport  Port=171
  VOUTP_HoodSW_flg : Outport  Port=172
  VOUTP_TailgateSW_flg : Outport  Port=173
  VOUTP_DrDoorSW_flg : Outport  Port=174
  VOUTP_PsDoorSW_flg : Outport  Port=175
  VOUTP_RLDoorSW_flg : Outport  Port=176
  VOUTP_RRDoorSW_flg : Outport  Port=177
  VOUTP_LockSetting_flg : Outport  Port=178
  VOUTP_FrChargingDoorCtrl_enum : Outport  Port=179
  VOUTP_RrChargingDoorCtrl_enum : Outport  Port=180
  VOUTP_CrashDetd_flg : Outport  Port=181
  VOUTP_CTDCtrl_enum : Outport  Port=182
  VOUTP_DoorLockIND_flg : Outport  Port=183
  VOUTP_CTDLockSW_flg : Outport  Port=184
  VOUTP_Dimmer_pct : Outport  Port=185
  VOUTP_DimmerEN_flg : Outport  Port=186
  VOUTP_PosLamp_flg : Outport  Port=187
  VOUTP_LBeam_flg : Outport  Port=188
  VOUTP_HBeam_flg : Outport  Port=189
  VOUTP_RrFogLamp_flg : Outport  Port=190
  VOUTP_BrakeLamp_flg : Outport  Port=191
  VOUTP_ReverseLamp_flg : Outport  Port=192
  VOUTP_LDRL_flg : Outport  Port=193
  VOUTP_RDRL_flg : Outport  Port=194
  VOUTP_LBSD_flg : Outport  Port=195
  VOUTP_RBSD_flg : Outport  Port=196
  VOUTP_HazardSW_flg : Outport  Port=197
  VOUTP_LTurnLP_flg : Outport  Port=198
  VOUTP_RTurnLP_flg : Outport  Port=199
  VOUTP_BCMBuzzerReq_flg : Outport  Port=200
  VOUTP_MirrorCtrl_enum : Outport  Port=201
  VOUTP_MirrorDefog_flg : Outport  Port=202
  VOUTP_RrDefog_flg : Outport  Port=203
  VOUTP_RoomLampH_flg : Outport  Port=204
  VOUTP_RoomLampL_flg : Outport  Port=205
  VOUTP_TrunkRel_flg : Outport  Port=206
  VOUTP_TailgateHDSW_flg : Outport  Port=207
  VOUTP_FrWiperL_flg : Outport  Port=208
  VOUTP_FrWiperH_flg : Outport  Port=209
  VOUTP_RrWiper_flg : Outport  Port=210
  VOUTP_WasherCtrl_enum : Outport  Port=211
  VOUTP_WiperFixMode_flg : Outport  Port=212
  VOUTP_User1DrAmbLightBrightness_enum : Outport  Port=213
  VOUTP_User1IPAmbLightBrightness_enum : Outport  Port=214
  VOUTP_User2DrAmbLightBrightness_enum : Outport  Port=215
  VOUTP_User2IPAmbLightBrightness_enum : Outport  Port=216
  VOUTP_User3DrAmbLightBrightness_enum : Outport  Port=217
  VOUTP_User3IPAmbLightBrightness_enum : Outport  Port=218
  VOUTP_User4DrAmbLightBrightness_enum : Outport  Port=219
  VOUTP_User4IPAmbLightBrightness_enum : Outport  Port=220
  VOUTP_User5DrAmbLightBrightness_enum : Outport  Port=221
  VOUTP_User5IPAmbLightBrightness_enum : Outport  Port=222
  VOUTP_User6DrAmbLightBrightness_enum : Outport  Port=223
  VOUTP_User6IPAmbLightBrightness_enum : Outport  Port=224
  VOUTP_User1AmbLightColor_enum : Outport  Port=225
  VOUTP_User2AmbLightColor_enum : Outport  Port=226
  VOUTP_User3AmbLightColor_enum : Outport  Port=227
  VOUTP_User4AmbLightColor_enum : Outport  Port=228
  VOUTP_User5AmbLightColor_enum : Outport  Port=229
  VOUTP_User6AmbLightColor_enum : Outport  Port=230
  VOUTP_AmbLightBreath1_flg : Outport  Port=231
  VOUTP_AmbLightBreath2_flg : Outport  Port=232
  VOUTP_AmbLightBreath3_flg : Outport  Port=233
  VOUTP_AmbLightBrightness1_enum : Outport  Port=234
  VOUTP_AmbLightBrightness2_enum : Outport  Port=235
  VOUTP_AmbLightBrightness3_enum : Outport  Port=236
  VOUTP_AmbLightColor1_enum : Outport  Port=237
  VOUTP_AmbLightColor2_enum : Outport  Port=238
  VOUTP_AmbLightColor3_enum : Outport  Port=239
  VOUTP_LampPwr_flg : Outport  Port=240
  VOUTP_SPTGDet_flg : Outport  Port=241
  VOUTP_APSOpenPTG_flg : Outport  Port=242
  VOUTP_FollowMe_flg : Outport  Port=243
  VOUTP_IVIRST_flg : Outport  Port=244
  VOUTP_CountAlarm_enum : Outport  Port=245
  VOUTP_MFSWTri_flg : Outport  Port=246
  VOUTP_MirrorFlodPos_flg : Outport  Port=247
  VOUTP_FuelDoorPos_flg : Outport  Port=248
  VOUTP_MFRDNBrightReq_pct : Outport  Port=249
  VOUTP_RoomLampMode_flg : Outport  Port=250
  VOUTP_IVIPTGUSStaSW_flg : Outport  Port=251
  VOUTP_PTGInnerSW2_enum : Outport  Port=252
  VOUTP_LDrvCtrlCmd_pct : Outport  Port=253
  VOUTP_LPasCtrlCmd_pct : Outport  Port=254
  VOUTP_LRLDCtrlCmd_pct : Outport  Port=255
  VOUTP_LRRDCtrlCmd_pct : Outport  Port=256
  VOUTP_APMDoorControlSta_flg : Outport  Port=257
  VOUTP_LockAlarm_enum : Outport  Port=258
  VOUTP_ATCtrl_enum : Outport  Port=259
  VOUTP_fUnlockSingle_flg : Outport  Port=260
  VOUTP_OutMode_enum : Outport  Port=261
  VOUTP_C3BMS6RCDTC_raw32 : Outport  Port=262
  VOUTP_C3BMS6CSDTC_raw32 : Outport  Port=263
  VOUTP_C3BMS6LCDTC_raw32 : Outport  Port=264
  VOUTP_C3BMS1RCDTC_raw32 : Outport  Port=265
  VOUTP_C3BMS1CSDTC_raw32 : Outport  Port=266
  VOUTP_C3BMS1LCDTC_raw32 : Outport  Port=267
  VOUTP_C3CCU1RCDTC_raw32 : Outport  Port=268
  VOUTP_C3CCU1CSDTC_raw32 : Outport  Port=269
  VOUTP_C3CCU1LCDTC_raw32 : Outport  Port=270
  VOUTP_C3CCU2RCDTC_raw32 : Outport  Port=271
  VOUTP_C3CCU2CSDTC_raw32 : Outport  Port=272
  VOUTP_C3CCU2LCDTC_raw32 : Outport  Port=273
  VOUTP_C1ABM1RCDTC_raw32 : Outport  Port=274
  VOUTP_C1ABM1CSDTC_raw32 : Outport  Port=275
  VOUTP_C1ABM1LCDTC_raw32 : Outport  Port=276
  VOUTP_Lv1ErrDTC_raw32 : Outport  Port=277
  VOUTP_Lv2ErrDTC_raw32 : Outport  Port=278
  VOUTP_Lv3ErrDTC_raw32 : Outport  Port=279
  VOUTP_Lv4ErrDTC_raw32 : Outport  Port=280
  VOUTP_BrkSWErrDTC_raw32 : Outport  Port=281
  VOUTP_BrkSWNoBacDTC_raw32 : Outport  Port=282
  VOUTP_KeyAuthDTC_raw32 : Outport  Port=283
  VOUTP_ONtoRdyDTC_raw32 : Outport  Port=284
  VOUTP_HVB4PreDTC_raw32 : Outport  Port=285
  VOUTP_MCU4PreDTC_raw32 : Outport  Port=286
  VOUTP_DCDC4PreDTC_raw32 : Outport  Port=287
  VOUTP_HVRlyCloDTC_raw32 : Outport  Port=288
  VOUTP_BMSRdyDTC_raw32 : Outport  Port=289
  VOUTP_DCDCEnaDTC_raw32 : Outport  Port=290
  VOUTP_HiLvSaChkDTC_raw32 : Outport  Port=291
  VOUTP_MidLvSaChkDTC_raw32 : Outport  Port=292
  VOUTP_MCUDisDTC_raw32 : Outport  Port=293
  VOUTP_DCDCDisDTC_raw32 : Outport  Port=294
  VOUTP_HVRlyOpDTC_raw32 : Outport  Port=295
  VOUTP_MCUActDTC_raw32 : Outport  Port=296
  VOUTP_OBC4PreDTC_raw32 : Outport  Port=297
  VOUTP_IniLVLoDTC_raw32 : Outport  Port=298
  VOUTP_LVSupLoDTC_raw32 : Outport  Port=299
  VOUTP_LVSupHiDTC_raw32 : Outport  Port=300
  VOUTP_DrStSWDTC_raw32 : Outport  Port=301
  VOUTP_FLDoorSWDTC_raw32 : Outport  Port=302
  VOUTP_RLDoorSWDTC_raw32 : Outport  Port=303
  VOUTP_FRDoorSWDTC_raw32 : Outport  Port=304
  VOUTP_RRDoorSWDTC_raw32 : Outport  Port=305
  VOUTP_HoodSWDTC_raw32 : Outport  Port=306
  VOUTP_TailgaSWDTC_raw32 : Outport  Port=307
  VOUTP_VehMalfunLevel_enum : Outport  Port=308
  VOUTP_APS1SigOoRDTC_raw32 : Outport  Port=309
  VOUTP_APS2SigOoRDTC_raw32 : Outport  Port=310
  VOUTP_APSCorrErrDTC_raw32 : Outport  Port=311
  VOUTP_MCUF1NoComDTC_raw32 : Outport  Port=312
  VOUTP_MCUR1NoComDTC_raw32 : Outport  Port=313
  VOUTP_Shifter1NoComDTC_raw32 : Outport  Port=314
  VOUTP_ESC7NoComDTC_raw32 : Outport  Port=315
  VOUTP_ESC1NoComDTC_raw32 : Outport  Port=316
  VOUTP_ESC5NoComDTC_raw32 : Outport  Port=317
  VOUTP_EnterNewOperCyc_flg : Outport  Port=318
  VOUTP_DiagHCrashDTC_raw32 : Outport  Port=319
  VOUTP_DiagFLTSDTC_raw32 : Outport  Port=320
  VOUTP_DiagFRTSDTC_raw32 : Outport  Port=321
  VOUTP_DiagRLTSDTC_raw32 : Outport  Port=322
  VOUTP_DiagRRTSDTC_raw32 : Outport  Port=323
  VOUTP_FCLUSSDTC_raw32 : Outport  Port=324
  VOUTP_FMLUSSDTC_raw32 : Outport  Port=325
  VOUTP_FMRUSSDTC_raw32 : Outport  Port=326
  VOUTP_FCRUSSDTC_raw32 : Outport  Port=327
  VOUTP_RCLUSSDTC_raw32 : Outport  Port=328
  VOUTP_RMLUSSDTC_raw32 : Outport  Port=329
  VOUTP_RMRUSSDTC_raw32 : Outport  Port=330
  VOUTP_RCRUSSDTC_raw32 : Outport  Port=331
  VOUTP_FLLUSSDTC_raw32 : Outport  Port=332
  VOUTP_FLRUSSDTC_raw32 : Outport  Port=333
  VOUTP_RLLUSSDTC_raw32 : Outport  Port=334
  VOUTP_RLRUSSDTC_raw32 : Outport  Port=335
  VOUTP_FCM2NoComDTC_raw32 : Outport  Port=336
  VOUTP_FCM2RCErrDTC_raw32 : Outport  Port=337
  VOUTP_FCM2CSErrDTC_raw32 : Outport  Port=338
  VOUTP_FCM3NoComDTC_raw32 : Outport  Port=339
  VOUTP_FCM3RCErrDTC_raw32 : Outport  Port=340
  VOUTP_FCM3CSErrDTC_raw32 : Outport  Port=341
  VOUTP_FCM4NoComDTC_raw32 : Outport  Port=342
  VOUTP_FCM4CSErrDTC_raw32 : Outport  Port=343
  VOUTP_FCM5NoComDTC_raw32 : Outport  Port=344
  VOUTP_FCM5CSErrDTC_raw32 : Outport  Port=345
  VOUTP_ZoneSCPNoComDTC_raw32 : Outport  Port=346
  VOUTP_BMSSigErrDetDTC_raw32 : Outport  Port=347
  VOUTP_FCMACCSigErrDetDTC_raw32 : Outport  Port=348
  VOUTP_FrMCUSigErrDetDTC_raw32 : Outport  Port=349
  VOUTP_RrMCUSigErrDetDTC_raw32 : Outport  Port=350
  VOUTP_CCUSigErrDetDTC_raw32 : Outport  Port=351
  VOUTP_ACCAccelCmdErrDetDTC_raw32 : Outport  Port=352
  VOUTP_ACCMalfuncDetDTC_raw32 : Outport  Port=353
  VOUTP_CCMalfuncDetDTC_raw32 : Outport  Port=354
  VOUTP_MSAMalfuncDetDTC_raw32 : Outport  Port=355
  VOUTP_ISAMalfuncDetDTC_raw32 : Outport  Port=356
  VOUTP_MCUF1RCErrDTC_raw32 : Outport  Port=357
  VOUTP_MCUR1RCErrDTC_raw32 : Outport  Port=358
  VOUTP_MCUF1CSErrDTC_raw32 : Outport  Port=359
  VOUTP_MCUR1CSErrDTC_raw32 : Outport  Port=360
  VOUTP_Shifter1RCErrDTC_raw32 : Outport  Port=361
  VOUTP_Shifter1CSErrDTC_raw32 : Outport  Port=362
  VOUTP_ESC7RCErrDTC_raw32 : Outport  Port=363
  VOUTP_ESC7CSErrDTC_raw32 : Outport  Port=364
  VOUTP_ESC1RCErrDTC_raw32 : Outport  Port=365
  VOUTP_ESC1CSErrDTC_raw32 : Outport  Port=366
  VOUTP_ESC5RCErrDTC_raw32 : Outport  Port=367
  VOUTP_ESC5CSErrDTC_raw32 : Outport  Port=368
  VOUTP_FrMCUTqErrDTC_raw32 : Outport  Port=369
  VOUTP_RrMCUTqErrDTC_raw32 : Outport  Port=370
  VOUTP_LFBatwarnDTC_raw32 : Outport  Port=371
  VOUTP_RFBatwarnDTC_raw32 : Outport  Port=372
  VOUTP_LRBatwarnDTC_raw32 : Outport  Port=373
  VOUTP_RRBatwarnDTC_raw32 : Outport  Port=374
  VOUTP_LFPressIndiDTC_raw32 : Outport  Port=375
  VOUTP_RFPressIndiDTC_raw32 : Outport  Port=376
  VOUTP_LRPressIndiDTC_raw32 : Outport  Port=377
  VOUTP_RRPressIndiDTC_raw32 : Outport  Port=378
  VOUTP_LFWheelTmpHighDTC_raw32 : Outport  Port=379
  VOUTP_RFWheelTmpHighDTC_raw32 : Outport  Port=380
  VOUTP_LRWheelTmpHighDTC_raw32 : Outport  Port=381
  VOUTP_RRWheelTmpHighDTC_raw32 : Outport  Port=382
  VOUTP_LFSensorFailDTC_raw32 : Outport  Port=383
  VOUTP_RFSensorFailDTC_raw32 : Outport  Port=384
  VOUTP_LRSensorFailDTC_raw32 : Outport  Port=385
  VOUTP_RRSensorFailDTC_raw32 : Outport  Port=386
  VOUTP_C1EPAS2LCDTC_raw32 : Outport  Port=387
  VOUTP_5vAPS1PwrErrDTC_raw32 : Outport  Port=388
  VOUTP_5vAPS2PwrErrDTC_raw32 : Outport  Port=389
  VOUTP_EPBLockTODTC_raw32 : Outport  Port=390
  VOUTP_EPBUnlockTODTC_raw32 : Outport  Port=391
  VOUTP_THCMAPTCWarning_raw32 : Outport  Port=392
  VOUTP_LimpHomeActTmp_flg : Outport  Port=393
  VOUTP_EDriveSysErr_VCUErrTmp_flg : Outport  Port=394
  VOUTP_ActAPSPosn_pct : Outport  Port=395
  VOUTP_EAPS1MIN_pct : Outport  Port=396
  VOUTP_EAPS2MIN_pct : Outport  Port=397
  VOUTP_DKCTimeSN_cnt : Outport  Port=398
  VOUTP_DKCAuthSta_enum : Outport  Port=399
  VOUTP_AllCANTxReq_flg : Outport  Port=400
  VOUTP_NMmTxReq_flg : Outport  Port=401
  VOUTP_Awake_enum : Outport  Port=402
  VOUTP_CSB_flg : Outport  Port=403
  VOUTP_ErrorState_enum : Outport  Port=404
  VOUTP_NodeID_enum : Outport  Port=405
  VOUTP_PNI_flg : Outport  Port=406
  VOUTP_RptMsgReq_flg : Outport  Port=407
  VOUTP_WakeUp_enum : Outport  Port=408
  VOUTP_ActiveWU_flg : Outport  Port=409
  VOUTP_SysNMmSta_enum : Outport  Port=410
  VOUTP_NetworkReq_flg : Outport  Port=411
  VOUTP_PowerUpState_enum : Outport  Port=412
  VOUTP_PowerDownState_enum : Outport  Port=413
  VOUTP_PowerUpFault_enum : Outport  Port=414
  VOUTP_PowerDownFault_enum : Outport  Port=415
  VOUTP_ActiveDischargeReq_flg : Outport  Port=416
  VOUTP_DCDCEnaReq_flg : Outport  Port=417
  VOUTP_DCDCVoltSetpoint_V : Outport  Port=418
  VOUTP_HVBatCnctReq_flg : Outport  Port=419
  VOUTP_HVSysReadyToCharge_enum : Outport  Port=420
  VOUTP_PowerSta_enum : Outport  Port=421
  VOUTP_LVPwrSta_flg : Outport  Port=422
  VOUTP_HVPwrSta_flg : Outport  Port=423
  VOUTP_SysPowerMode_enum : Outport  Port=424
  VOUTP_FrMCUEnaReq_flg : Outport  Port=425
  VOUTP_RrMCUEnaReq_flg : Outport  Port=426
  VOUTP_DrivetrainSelect_enum : Outport  Port=427
  VOUTP_DrSeatSta_enum : Outport  Port=428
  VOUTP_PwrStaSelect_enum : Outport  Port=429
  VOUTP_PwrStaConstraint_enum : Outport  Port=430
  VOUTP_TCountSta_enum : Outport  Port=431
  VOUTP_PwrUpReq_enum : Outport  Port=432
  VOUTP_PwrDownReq_enum : Outport  Port=433
  VOUTP_LowSOCWarn_enum : Outport  Port=434
  VOUTP_ReVehThdChkSta_enum : Outport  Port=435
  VOUTP_LVSysErrPwrOutErr_flg : Outport  Port=436
  VOUTP_EvccAplusPwrUpReq_flg : Outport  Port=437
  VOUTP_PwrStaONTOPopReq_flg : Outport  Port=438
  VOUTP_IVIPwrStaONTOPopT_s : Outport  Port=439
  VOUTP_LVChrgHoldTtimer_s : Outport  Port=440
  VOUTP_LVBattChrgTimeCnt_s : Outport  Port=441
  VOUTP_SilentChkAllowSleep_flg : Outport  Port=442
  VOUTP_TimerAllowSleep_flg : Outport  Port=443
  VOUTP_FDADC12VDetAvg_mV : Outport  Port=444
  VOUTP_PMMAllowECUSleep_flg : Outport  Port=445
  VOUTP_LVSilentChrgSta_enum : Outport  Port=446
  VOUTP_LVSilentChrgReq_flg : Outport  Port=447
  VOUTP_LVSilentChrgLv_enum : Outport  Port=448
  VOUTP_CtrlFrPwrStbA1P_flg : Outport  Port=449
  VOUTP_CtrlFrRC1_flg : Outport  Port=450
  VOUTP_CtrlFrBMSCCUCIR_flg : Outport  Port=451
  VOUTP_CtrlFrEDUINVERTER_flg : Outport  Port=452
  VOUTP_HWResetSta_enum : Outport  Port=453
  VOUTP_CtrlDrPwrStbA2_flg : Outport  Port=454
  VOUTP_PwrStaTOSta_enum : Outport  Port=455
  VOUTP_Sched_ChgTOSta_enum : Outport  Port=456
  VOUTP_PwrReq_OTA_enum : Outport  Port=457
  VOUTP_OTAPwrReqOFFChkSta_enum : Outport  Port=458
  VOUTP_OTAPwrReqStdChkSta_enum : Outport  Port=459
  VOUTP_HWVer1_cnt : Outport  Port=460
  VOUTP_HWVer2_cnt : Outport  Port=461
  VOUTP_HWVer3_cnt : Outport  Port=462
  VOUTP_CarModel1_cnt : Outport  Port=463
  VOUTP_CarModel2_cnt : Outport  Port=464
  VOUTP_CarModel3_cnt : Outport  Port=465
  VOUTP_ECU1_cnt : Outport  Port=466
  VOUTP_ECU2_cnt : Outport  Port=467
  VOUTP_Major1_cnt : Outport  Port=468
  VOUTP_Major2_cnt : Outport  Port=469
  VOUTP_Minor1_cnt : Outport  Port=470
  VOUTP_Minor2_cnt : Outport  Port=471
  VOUTP_Patch1_cnt : Outport  Port=472
  VOUTP_Patch2_cnt : Outport  Port=473
  VOUTP_Country1_cnt : Outport  Port=474
  VOUTP_Country2_cnt : Outport  Port=475
  VOUTP_Variation_cnt : Outport  Port=476
  VOUTP_Dash1_cnt : Outport  Port=477
  VOUTP_Change1_cnt : Outport  Port=478
  VOUTP_Change2_cnt : Outport  Port=479
  VOUTP_Dash2_cnt : Outport  Port=480
  VOUTP_SHA1_cnt : Outport  Port=481
  VOUTP_SHA2_cnt : Outport  Port=482
  VOUTP_SHA3_cnt : Outport  Port=483
  VOUTP_SHA4_cnt : Outport  Port=484
  VOUTP_SHA5_cnt : Outport  Port=485
  VOUTP_SHA6_cnt : Outport  Port=486
  VOUTP_SHA7_cnt : Outport  Port=487
  VOUTP_SHA8_cnt : Outport  Port=488
  VOUTP_NvWriteReqRisingEdge_flg : Outport  Port=489
  VOUTP_FdcSlpReqRisingEdge_flg : Outport  Port=490
  VOUTP_FdcSlpTime_sec : Outport  Port=491
  VOUTP_PmicBootReason_enum : Outport  Port=492
  VOUTP_WisrBootReason_raw32 : Outport  Port=493
  VOUTP_AcoreRebootCmdACK_flg : Outport  Port=494
  VOUTP_CurrentNmState_enum : Outport  Port=495
  VOUTP_FDCompCmd_rpm : Outport  Port=496
  VOUTP_FDSOV1Cmd_flg : Outport  Port=497
  VOUTP_FDSOV2Cmd_flg : Outport  Port=498
  VOUTP_FDSOV3Cmd_flg : Outport  Port=499
  VOUTP_FDEXV1Cmd_step : Outport  Port=500
  VOUTP_FDEXV2Cmd_step : Outport  Port=501
  VOUTP_FDSOTXVCmd_flg : Outport  Port=502
  VOUTP_FDFWVCmd_flg : Outport  Port=503
  VOUTP_FDTWVCmd_pct : Outport  Port=504
  VOUTP_FDFrWPTCHeatPwrCmd_W : Outport  Port=505
  VOUTP_CoolgFanActDuty_pct : Outport  Port=506
  VOUTP_FDAGSCmd_enum : Outport  Port=507
  VOUTP_FDEWP1Cmd_enum : Outport  Port=508
  VOUTP_FDEWP2Cmd_enum : Outport  Port=509
  VOUTP_FDEWP3Cmd_enum : Outport  Port=510
  VOUTP_FDFrLeAPTCHeatPwrCmd_W : Outport  Port=511
  VOUTP_FDFrRiAPTCHeatPwrCmd_W : Outport  Port=512
  VOUTP_FDRrAPTCHeatPwrCmd_W : Outport  Port=513
  VOUTP_FDBlowerCmd_pct : Outport  Port=514
  VOUTP_BatteryMode_enum : Outport  Port=515
  VOUTP_EDriveMode_enum : Outport  Port=516
  VOUTP_CabinMode_enum : Outport  Port=517
  VOUTP_CCUACLampSts_flg : Outport  Port=518
  VOUTP_CCUAutoLampSts_flg : Outport  Port=519
  VOUTP_CCUACMaxLampSts_flg : Outport  Port=520
  VOUTP_CCUSyncLampSts_flg : Outport  Port=521
  VOUTP_sigAirIntenZon1St_enum : Outport  Port=522
  VOUTP_sigWindDirZon1St_enum : Outport  Port=523
  VOUTP_sigRecircSt_flg : Outport  Port=524
  VOUTP_sigSetTempZon1St_C : Outport  Port=525
  VOUTP_sigSetTempZon2St_C : Outport  Port=526
  VOUTP_sigClntTHvBattOut_C : Outport  Port=527
  VOUTP_sigCbnSolarLeft_W : Outport  Port=528
  VOUTP_sigClntTHvBattIn_C : Outport  Port=529
  VOUTP_sigCbnSolarRight_W : Outport  Port=530
  VOUTP_sigAmbAirT_C : Outport  Port=531
  VOUTP_sigCbnAirT_C : Outport  Port=532
  VOUTP_ACSubMode_enum : Outport  Port=533
  VOUTP_FDRecyAutoCmd_enum : Outport  Port=534
  VOUTP_ACModeMem_enum : Outport  Port=535
  VOUTP_Face_flg : Outport  Port=536
  VOUTP_Foot_flg : Outport  Port=537
  VOUTP_Frost_flg : Outport  Port=538
  VOUTP_FaceM_flg : Outport  Port=539
  VOUTP_FootM_flg : Outport  Port=540
  VOUTP_CCUSyncSts_flg : Outport  Port=541
  VOUTP_ACForceOFF_flg : Outport  Port=542
  VOUTP_RecAutoFlg_flg : Outport  Port=543
  VOUTP_AirIntenZone1M_enum : Outport  Port=544
  VOUTP_fdefog_flg : Outport  Port=545
  VOUTP_sigSetTempZon2StM_C : Outport  Port=546
  VOUTP_sigDfrstSt_flg : Outport  Port=547
  VOUTP_FDCTHCAirIntZ3Sta_enum : Outport  Port=548
  VOUTP_FDCTHCDrEVentModeSta_enum : Outport  Port=549
  VOUTP_FDCTHCPsEVentModeSta_enum : Outport  Port=550
  VOUTP_FDCTHCDrEVentZSta_enum : Outport  Port=551
  VOUTP_FDCTHCCLEVentZSta_enum : Outport  Port=552
  VOUTP_FDCTHCPsEVentZSta_enum : Outport  Port=553
  VOUTP_FDCTHCCREVentZSta_enum : Outport  Port=554
  VOUTP_FDCTHCDrEVentYSta_enum : Outport  Port=555
  VOUTP_FDCTHCDrVentENSta_flg : Outport  Port=556
  VOUTP_FDCTHCCLEVentYSta_enum : Outport  Port=557
  VOUTP_FDCTHCCLVentENSta_flg : Outport  Port=558
  VOUTP_FDCTHCPsEVentYSta_enum : Outport  Port=559
  VOUTP_FDCTHCPsVentENSta_flg : Outport  Port=560
  VOUTP_FDCTHCCREVentYSta_enum : Outport  Port=561
  VOUTP_FDCTHCCRVentENSta_flg : Outport  Port=562
  VOUTP_FDCTHCMAPTCForceOFFSta_flg : Outport  Port=563
  VOUTP_DrVentEN_flg : Outport  Port=564
  VOUTP_CLVentEN_flg : Outport  Port=565
  VOUTP_PsVentEN_flg : Outport  Port=566
  VOUTP_CRVentEN_flg : Outport  Port=567
  VOUTP_FDCFGSAirIntSta_enum : Outport  Port=568
  VOUTP_FDCFGSChSta_enum : Outport  Port=569
  VOUTP_FDCFGSAirIntCmd_enum : Outport  Port=570
  VOUTP_FDCFGSFuncSta_flg : Outport  Port=571
  VOUTP_FDCFGSChCmd_enum : Outport  Port=572
  VOUTP_FDCFGSIONSWSta_flg : Outport  Port=573
  VOUTP_FDCFGSIONCmd_flg : Outport  Port=574
  VOUTP_FDCFGSLearnCmd_enum : Outport  Port=575
  VOUTP_FDCTHCMPreWPTCHeatSta_enum : Outport  Port=576
  VOUTP_LFBatWarn_flg : Outport  Port=577
  VOUTP_RFBatWarn_flg : Outport  Port=578
  VOUTP_LRBatWarn_flg : Outport  Port=579
  VOUTP_RRBatWarn_flg : Outport  Port=580
  VOUTP_LFWheelPress_raw8 : Outport  Port=581
  VOUTP_RFWheelPress_raw8 : Outport  Port=582
  VOUTP_LRWheelPress_raw8 : Outport  Port=583
  VOUTP_RRWheelPress_raw8 : Outport  Port=584
  VOUTP_LFWheelTemp_C : Outport  Port=585
  VOUTP_RFWheelTemp_C : Outport  Port=586
  VOUTP_LRWheelTemp_C : Outport  Port=587
  VOUTP_RRWheelTemp_C : Outport  Port=588
  VOUTP_LFSensorFail_flg : Outport  Port=589
  VOUTP_RFSensorFail_flg : Outport  Port=590
  VOUTP_LRSensorFail_flg : Outport  Port=591
  VOUTP_RRSensorFail_flg : Outport  Port=592
